simulink model "IEEE_34_node_2020a_scenarios_fold"  (R2020a)
settings: Solver=FixedStepDiscrete  StartTime=0.0  StopTime=0.001  RelTol=1e-3
InitFcn:
  | power_34NodeTestFeeder_init;
  | %=============================
  | Vnom_ph_ph = 24900;
  | Vnom = 24900/sqrt(3);
  | Vnom1_ph_ph = 4160;
  | Vnom1 = 4160/sqrt(3);
  | Degrees_ph_ph_gen1 = 0;
  | Frequency = 60;
  | Apparent_power_gen1 = 2500e3;
  | base_current=1.5e6;
  | SW850_816=1;
  | SW818_820=1;
  | SW832_858=1;
  | SW834_842=1;
  | SW836_862=1;
  | %=============================
  | %824-828===Load1=================
  | V_824_828 = [1.008 1.016 1.012];
  | Pa_824_828 = [1e-6 1e-6 4]*1e3*1;
  | Pp_824_828 = [1e-6 1e-6 2]*1e3*1;
  | Pn_824_828 = [1e-6 1e-6 1e-6]*1;
  | 
  | %820-822===Load2=================
  | V_820_822 = 0.993;
  | Pa_820_822 = 135e3*1;
  | Pp_820_822 = 70e3*1;
  | Pn_820_822 = 1e-6*1;
  | 
  | %858-834===Load3=================
  | V_858_834 = [1.034 1.032 1.034]*sqrt(3);
  | Pa_858_834 = [4 15 13]*1e3*1;
  | Pp_858_834 = [2 8 7]*1e3*1;
  | Pn_858_834 = [1e-6 1e-6 1e-6]*1;
  | 
  | %844 B.V.c===Load4================
  | V_844 = [1.031 1.029 1.031];
  | Pa_844 = [135 135 135]*1e3*1;
  | Pp_844 = [105 105 105]*1e3*1;
  | Pn_844 = [100 100 100]*1e3*1;
  | 
  | %840======Load5=================
  | V_840 = [1.03 1.029 1.031];
  | Pa_840 = [9 9 9]*1e3*1;
  | Pp_840 = [7 7 7]*1e3*1;
  | Pn_840 = [1e-6 1e-6 1e-6]*1;
  | 
  | % For Distributed Loads==================================================
  | %802-806
  | V_802_806 = [1.047 1.048 1.048];
  | Pa_802_806 = [1e-6 30 25]*1e3;
  | Pp_802_806 = [1e-6 15 14]*1e3;
  | Pn_802_806 = [1e-6 1e-6 1e-6];
  | 
  | %808-810
  | V_808_810 = 1.014;
  | Pa_808_810 = 16e3;
  | Pp_808_810 = 8e3;
  | Pn_808_810 = 1e-6;
  | 
  | %816-824
  | V_816_824 = [1.017 1.025 1.02]*sqrt(3);
  | Pa_816_824 = [1e-6 5 1e-6]*1e3;
  | Pp_816_824 = [1e-6 2 1e-6]*1e3;
  | Pn_816_824 = [1e-6 1e-6 1e-6];
  | 
  | %818-820
  | V_818_820 = 1.016;
  | Pa_818_820 = 34e3;
  | Pp_818_820 = 17e3;
  | Pn_818_820 = 1e-6;
  | 
  | %824-826
  | V_824_826 = 1.008;
  | Pa_824_826 = 40e3;
  | Pp_824_826 = 20e3;
  | Pn_824_826 = 1e-6;
  | 
  | %828-830
  | V_828_830 = [1.007 1.015 1.011];
  | Pa_828_830 = [7 1e-6 1e-6]*1e3;
  | Pp_828_830 = [3 1e-6 1e-6]*1e3;
  | Pn_828_830 = [1e-6 1e-6 1e-6];
  | 
  | %832-858
  | V_832_858 = [1.036 1.035 1.036]*sqrt(3);
  | Pa_832_858 = [7 2 6]*1e3;
  | Pp_832_858 = [3 1 3]*1e3;
  | Pn_832_858 = [1e-6 1e-6 1e-6];
  | 
  | %834-860
  | V_834_860 = [1.031 1.029 1.031]*sqrt(3);
  | Pa_834_860 = [16 20 110]*1e3;
  | Pp_834_860 = [8 10 55]*1e3;
  | Pn_834_860 = [1e-6 1e-6 1e-6];
  | 
  | %836-840
  | V_836_840 = [1.03 1.029 1.031]*sqrt(3);
  | Pa_836_840 = [18 22 1e-6]*1e3;
  | Pp_836_840 = [9 11 1e-6]*1e3;
  | Pn_836_840 = [1e-6 1e-6 1e-6];
  | 
  | %842-844
  | V_842_844 = [1.031 1.029 1.031];
  | Pa_842_844 = [9 1e-6 1e-6]*1e3;
  | Pp_842_844 = [5 1e-6 1e-6]*1e3;
  | Pn_842_844 = [1e-6 1e-6 1e-6];
  | 
  | %844-846
  | V_844_846 = [1.031 1.029 1.031];
  | Pa_844_846 = [1e-6 25 20]*1e3;
  | Pp_844_846 = [1e-6 12 11]*1e3;
  | Pn_844_846 = [1e-6 1e-6 1e-6];
  | 
  | %846-848
  | V_846_848 = [1.031 1.029 1.031];
  | Pa_846_848 = [1e-6 23 1e-6]*1e3;
  | Pp_846_848 = [1e-6 11 1e-6]*1e3;
  | Pn_846_848 = [1e-6 1e-6 1e-6];
  | 
  | %854-856
  | V_854_856 = 0.998;
  | Pa_854_856 = 4e3;
  | Pp_854_856 = 2e3;
  | Pn_854_856 = 1e-6;
  | 
  | %858-864
  | V_858_864 = 1.034;
  | Pa_858_864 = 2e3;
  | Pp_858_864 = 1e3;
  | Pn_858_864 = 1e-6;
  | 
  | %860-836
  | V_860_836 = [1.03 1.029 1.031]*sqrt(3);
  | Pa_860_836 = [30 10 42]*1e3;
  | Pp_860_836 = [15 6 22]*1e3;
  | Pn_860_836 = [1e-6 1e-6 1e-6];
  | 
  | %862-838
  | V_862_838 = 1.029;
  | Pa_862_838 = 28e3;
  | Pp_862_838 = 14e3;
  | Pn_862_838 = 1e-6;
  | 
  | % For Spot Loads===========================================================
  | %830
  | V_830 = [0.989 0.998 0.994]*sqrt(3);
  | Pa_830 = [10 10 25]*1e3;
  | Pp_830 = [5 5 10]*1e3;
  | Pn_830 = [1e-6 1e-6 1e-6];
  | 
  | %848 B.V.c
  | V_848 = [1.031 1.029 1.031]*sqrt(3);
  | Pa_848 = [20 20 20]*1e3;
  | Pp_848 = [16 16 16]*1e3;
  | Pn_848 = [150 150 150]*1e3;
  | 
  | %860
  | V_860 = [1.03 1.029 1.031];
  | Pa_860 = [20 20 20]*1e3;
  | Pp_860 = [16 16 16]*1e3;
  | Pn_860 = [1e-6 1e-6 1e-6];
  | 
  | %890
  | V_890 = [0.917 0.924 0.918]*sqrt(3);
  | Pa_890 = [150 150 150]*1e3;
  | Pp_890 = [75 75 75]*1e3;
  | Pn_890 = [1e-6 1e-6 1e-6];
undefined symbols (not defined in the file or in its folder): Angle, C_300, C_301, C_302, C_303, C_304, Degrees_ph, ft2km, L_300, L_301, L_302, L_303, L_304, Magnitude, ph, ph_gen1, R_300, R_301, R_302, R_303, R_304, Vnom_ph
libraries: powerlib x177
(part 1 of 2)
settings Model: Creator=liyifu  LastModifiedBy=l4729
settings DataIOCC: ReturnWorkspaceOutputs=off
settings DebuggingCC: ArithmeticOperatorsInVariantConditions=warning
settings SFSimCC: SimUseLocalCustomCode=off  CustomCodeUndefinedFunction=UseInterfaceOnly
settings RTWCC: RTWUseLocalCustomCode=off

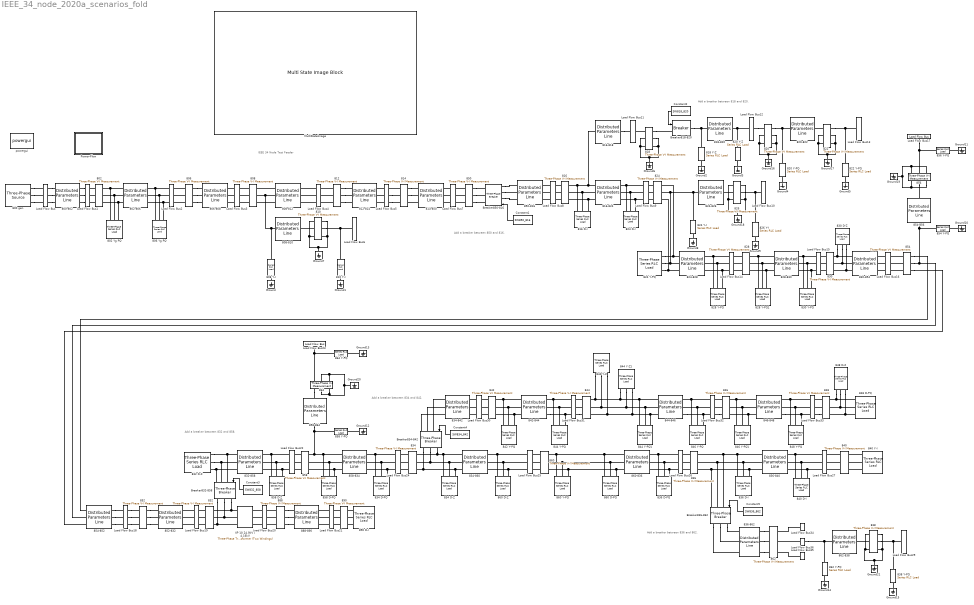
== system IEEE_34_node_2020a_scenarios_fold ==
  note: Add a breaker between 832 and 858.
  note: IEEE 34 Node Test Feeder
  note: Add a breaker between 834 and 842.
  note: Add a breaker between 836 and 862.
  note: Add a breaker between 850 and 816.
  note: Add a breaker between 818 and 820.
  800 gen : powerlib/Electrical Sources/Three-Phase Source  InternalConnection=Yg  VoltagePhases=on  Voltage=Vnom_ph-ph  PhaseAngle=Degrees_ph-ph_gen1  Voltage_phases=[1.05 1.05 1.05]*Vnom  PhaseAngles_phases=[0 -120 +120]  Frequency=Frequency  NonIdealSource=off  SpecifyImpedance=on  Resistance=0.8929  Inductance=16.58e-3  ShortCircuitLevel=Apparent_power_gen1  BaseVoltage=Vnom_ph_ph  XRratio=8  BusType=swing  Pref=10e3  Qref=0  Prefabc=[10e3, 10e3, 10e3]  Qrefabc=[0, 0, 0]  Qmin=-inf  Qmax=inf
  800-802 : powerlib/Elements/Distributed Parameters Line  Phases=3  Frequency=Frequency  Resistance=R_300  Inductance=L_300  Capacitance=C_300  Length=2580*ft2km  x1=[1249.92108084395 26131.4308609001 26009.0181767455;376.991118430775 376.991118430775 376.991118430775;1.94160573810255 0.298080075052811 1.87234868535801]  x2=[1257.86990495326 26107.3117545713 25983.4479681992;376.991118430775 376.991118430775 376.991118430775;1.93807520662352 0.296564075731698 1.87075709202379]  x3=[7.13297479988852 32.3957031974537 23.1415422380633;376.991118430775 376.991118430775 376.991118430775;0.709542259543237 -0.812774214222377 0.255094598667959]  x4=[6.75296406809703 144.806609038061 132.501806105152;376.991118430775 376.991118430775 376.991118430775;-2.86917677084019 0.498468146483693 2.04637828745182]  x5=3.46223763231864e-06  V1=ones(3,3)  V2=ones(3,3)  I1=ones(3,3)  I2=ones(3,3)  nHarmo=1  Measurements=None
  802 : powerlib/Measurements/Three-Phase V-I Measurement  VoltageMeasurement=phase-to-ground  SetLabelV=on  LabelV=Vabc_802  Vpu=on  VpuLL=off  CurrentMeasurement=yes  SetLabelI=on  LabelI=Iabc_802  Ipu=on  Pbase=base_current  Vbase=Vnom_ph_ph  OutputType=Magnitude-Angle  PhasorSimulation=on  PSBequivalent=0
  802 Yg PQ : powerlib/Elements/Three-Phase Series RLC Load  LConnTagsString=A|B|C  Configuration=Y (grounded)  NominalVoltage=[  Vabc=V_802_806*Vnom  Vabcp=[1e3 1e3 1e3]  NominalFrequency=Frequency  UnbalancedPower=on  ActivePower=10e3  InductivePower=100  CapacitivePower=100  Pabc=Pa_802_806/2  QLabc=Pp_802_806/2  QCabc=Pn_802_806  Pabcp=[10e3 9e3 11e3]  QLabcp=[100 90 110]  QCabcp=[100 90 110]  Measurements=None  LoadType=constant PQ
      settings: AttributesFormatString=|
      | P= %<Pabc> W
      | Ql=%<QLabc> var
      | Qc=%<QCabc> var
  802-806 : powerlib/Elements/Distributed Parameters Line  Phases=3  Frequency=Frequency  Resistance=R_300  Inductance=L_300  Capacitance=C_300  Length=1730*ft2km  x1=[1257.86990495326 26107.3117545713 25983.4479681992;376.991118430775 376.991118430775 376.991118430775;1.93850522519394 0.296930576358522 1.87111645643134]  x2=[1263.00777604381 26091.4526622714 25967.1255164436;376.991118430775 376.991118430775 376.991118430775;1.93674169452962 0.295921998479355 1.87004589016608]  x3=[6.73268295673131 32.7537595825314 24.3418370556638;376.991118430775 376.991118430775 376.991118430775;0.817345362469665 -0.791135380998958 0.306817144760857]  x4=[6.06072552939003 143.954163081489 131.457799242515;376.991118430775 376.991118430775 376.991118430775;-2.79432744429802 0.498877931254703 2.05645367118062]  x5=2.32157794725242e-06  V1=ones(3,3)  V2=ones(3,3)  I1=ones(3,3)  I2=ones(3,3)  nHarmo=1  Measurements=None
  806 : powerlib/Measurements/Three-Phase V-I Measurement  VoltageMeasurement=phase-to-ground  SetLabelV=on  LabelV=Vabc_806  Vpu=on  VpuLL=off  CurrentMeasurement=yes  SetLabelI=on  LabelI=Iabc_806  Ipu=on  Pbase=base_current  Vbase=Vnom_ph_ph  OutputType=Magnitude-Angle  PhasorSimulation=on  PSBequivalent=0
  806 Yg PQ : powerlib/Elements/Three-Phase Series RLC Load  LConnTagsString=A|B|C  Configuration=Y (grounded)  NominalVoltage=[  Vabc=V_802_806*Vnom  Vabcp=[1e3 1e3 1e3]  NominalFrequency=Frequency  UnbalancedPower=on  ActivePower=10e3  InductivePower=100  CapacitivePower=100  Pabc=Pa_802_806/2  QLabc=Pp_802_806/2  QCabc=Pn_802_806  Pabcp=[10e3 9e3 11e3]  QLabcp=[100 90 110]  QCabcp=[100 90 110]  Measurements=None  LoadType=constant PQ
      settings: AttributesFormatString=|
      | P= %<Pabc> W
      | Ql=%<QLabc> var
      | Qc=%<QCabc> var
  806-808 : powerlib/Elements/Distributed Parameters Line  Phases=3  Frequency=Frequency  Resistance=R_300  Inductance=L_300  Capacitance=C_300  Length=32230*ft2km  x1=[1263.00777604381 26091.4526622714 25967.1255164436;376.991118430775 376.991118430775 376.991118430775;1.92131161641447 0.282771093634514 1.85715104965965]  x2=[1355.16892465068 25803.6960566382 25680.9632225794;376.991118430775 376.991118430775 376.991118430775;1.90095381776325 0.264070563711962 1.8370468229557]  x3=[6.3768548007228 32.6175711680747 25.3697798294854;376.991118430775 376.991118430775 376.991118430775;0.920439308030638 -0.792962958654931 0.330886039817891]  x4=[5.31865755565328 140.041353428377 128.050295750342;376.991118430775 376.991118430775 376.991118430775;-2.73456087382505 0.471033237587638 2.03937541131982]  x5=4.32511313525697e-05  V1=ones(3,3)  V2=ones(3,3)  I1=ones(3,3)  I2=ones(3,3)  nHarmo=1  Measurements=None
  808 : powerlib/Measurements/Three-Phase V-I Measurement  VoltageMeasurement=phase-to-ground  SetLabelV=on  LabelV=Vabc_808  Vpu=on  VpuLL=off  CurrentMeasurement=yes  SetLabelI=on  LabelI=Iabc_808  Ipu=on  Pbase=base_current  Vbase=Vnom_ph_ph  OutputType=Magnitude-Angle  PhasorSimulation=on  PSBequivalent=0
  808 Y-I : powerlib/Elements/Series RLC Load  LConnTagsString=a  RConnTagsString=__new0  NominalVoltage=V_808_810*Vnom  NominalFrequency=Frequency  ActivePower=Pa_808_810/2  InductivePower=Pp_808_810/2  CapacitivePower=Pn_808_810  Setx0=off  InitialVoltage=0  SetiL0=off  InitialCurrent=0  Measurements=None  LoadType=constant I
      settings: AttributesFormatString=|
      | P=%<ActivePower> W
      | Ql=%<InductivePower> var
      | Qc=%<CapacitivePower> var
  808-810 : powerlib/Elements/Distributed Parameters Line  Phases=1  Frequency=Frequency  Resistance=R_303(2,2)  Inductance=L_303(2,2)  Capacitance=C_303(2,2)  Length=5804*ft2km  x1=[21047.5384749886;376.991118430775;-2.12176362657333]  x2=[21044.5333181041;376.991118430775;-2.12177432032583]  x3=[34.5695272211914;376.991118430775;-2.11315403228961]  x4=[36.1457970114117;376.991118430775;-2.13270557006442]  x5=7.30496713110932e-06  V1=ones(3,3)  V2=ones(3,3)  I1=ones(3,3)  I2=ones(3,3)  nHarmo=1  Measurements=None
  808-812 : powerlib/Elements/Distributed Parameters Line  Phases=3  Frequency=Frequency  Resistance=R_300  Inductance=L_300  Capacitance=C_300  Length=37500*ft2km  x1=[1355.16892465068 25803.6960566382 25680.9632225794;376.991118430775 376.991118430775 376.991118430775;1.89828770262664 0.261798259825657 1.83481876362885]  x2=[1443.44628212571 25479.8515014695 25364.0620665995;376.991118430775 376.991118430775 376.991118430775;1.88295137638678 0.240192551529379 1.81094740401628]  x3=[5.46905993850028 32.6245925749511 26.6761925732301;376.991118430775 376.991118430775 376.991118430775;0.995018334108287 -0.794161100185234 0.309761347978168]  x4=[4.23685935060835 137.208461244538 126.419269863165;376.991118430775 376.991118430775 376.991118430775;-2.8061655132456 0.449094607298641 2.02713913226157]  x5=5.03232213999802e-05  V1=ones(3,3)  V2=ones(3,3)  I1=ones(3,3)  I2=ones(3,3)  nHarmo=1  Measurements=None
  810 : powerlib/Measurements/Three-Phase V-I Measurement  VoltageMeasurement=phase-to-ground  SetLabelV=on  LabelV=Vabc_810  Vpu=on  VpuLL=off  CurrentMeasurement=yes  SetLabelI=on  LabelI=Iabc_810  Ipu=on  Pbase=base_current  Vbase=Vnom_ph_ph  OutputType=Magnitude-Angle  PhasorSimulation=on  PSBequivalent=0
  810 Y-I : powerlib/Elements/Series RLC Load  LConnTagsString=a  RConnTagsString=__new0  NominalVoltage=V_808_810*Vnom  NominalFrequency=Frequency  ActivePower=Pa_808_810/2  InductivePower=Pp_808_810/2  CapacitivePower=Pn_808_810  Setx0=off  InitialVoltage=0  SetiL0=off  InitialCurrent=0  Measurements=None  LoadType=constant I
      settings: AttributesFormatString=|
      | P=%<ActivePower> W
      | Ql=%<InductivePower> var
      | Qc=%<CapacitivePower> var
  812 : powerlib/Measurements/Three-Phase V-I Measurement  VoltageMeasurement=phase-to-ground  SetLabelV=on  LabelV=Vabc_812  Vpu=on  VpuLL=off  CurrentMeasurement=yes  SetLabelI=on  LabelI=Iabc_812  Ipu=on  Pbase=base_current  Vbase=Vnom_ph_ph  OutputType=Magnitude-Angle  PhasorSimulation=on  PSBequivalent=0
  812-814 : powerlib/Elements/Distributed Parameters Line  Phases=3  Frequency=Frequency  Resistance=R_300  Inductance=L_300  Capacitance=C_300  Length=29730*ft2km  x1=[1443.44628212571 25479.8515014695 25364.0620665995;376.991118430775 376.991118430775 376.991118430775;1.88688225202464 0.243542798435754 1.814232417483]  x2=[1513.27779103294 25226.8818502461 25118.6711360678;376.991118430775 376.991118430775 376.991118430775;1.87617344887056 0.226298980649994 1.79510755585285]  x3=[5.53984525286875 32.6362598627681 27.1978990110373;376.991118430775 376.991118430775 376.991118430775;1.01474929706559 -0.819913423956052 0.285686013441521]  x4=[4.19567507962093 136.436942339818 125.720705102048;376.991118430775 376.991118430775 376.991118430775;-2.82219411836218 0.437343389389646 2.01609371330485]  x5=3.98962499259043e-05  V1=ones(3,3)  V2=ones(3,3)  I1=ones(3,3)  I2=ones(3,3)  nHarmo=1  Measurements=None
  814 : powerlib/Measurements/Three-Phase V-I Measurement  VoltageMeasurement=phase-to-ground  SetLabelV=on  LabelV=Vabc_814  Vpu=on  VpuLL=off  CurrentMeasurement=yes  SetLabelI=on  LabelI=Iabc_814  Ipu=on  Pbase=base_current  Vbase=Vnom_ph_ph  OutputType=Magnitude-Angle  PhasorSimulation=on  PSBequivalent=0
  814-850 : powerlib/Elements/Distributed Parameters Line  Phases=3  Frequency=Frequency  Resistance=R_301  Inductance=L_301  Capacitance=C_301  Length=10*ft2km  x1=[749.994335266099 25229.1164810927 25142.5492609672;376.991118430775 376.991118430775 376.991118430775;-0.624184699531901 0.237600670627926 1.80412447902211]  x2=[749.971210173394 25228.9677045473 25142.4037426608;376.991118430775 376.991118430775 376.991118430775;-0.624161374265916 0.237593581391487 1.80411674762356]  x3=[4.46442861433734 31.9624950383377 28.1850985340397;376.991118430775 376.991118430775 376.991118430775;0.862042492492586 -0.884382499448575 0.236346932718508]  x4=[4.62367269240938 136.132716168199 125.203043967645;376.991118430775 376.991118430775 376.991118430775;-1.91880432400362 0.45074101824152 2.03117866069587]  x5=1.37899021776565e-08  V1=ones(3,3)  V2=ones(3,3)  I1=ones(3,3)  I2=ones(3,3)  nHarmo=1  Measurements=None
  816 : powerlib/Measurements/Three-Phase V-I Measurement  VoltageMeasurement=phase-to-ground  SetLabelV=on  LabelV=Vabc_816  Vpu=on  VpuLL=off  CurrentMeasurement=yes  SetLabelI=on  LabelI=Iabc_816  Ipu=on  Pbase=base_current  Vbase=Vnom_ph_ph  OutputType=Magnitude-Angle  PhasorSimulation=on  PSBequivalent=0
  816 D-I : powerlib/Elements/Three-Phase Series RLC Load  LConnTagsString=A|B|C  Configuration=Delta  NominalVoltage=[  Vabc=[1.017 1.025 1.02]*sqrt(3)*Vnom  Vabcp=V_816_824*Vnom  NominalFrequency=Frequency  UnbalancedPower=on  ActivePower=10e3  InductivePower=100  CapacitivePower=100  Pabc=[0 30 25]*1e3/2  QLabc=[0 15 14]*1e3/2  QCabc=[0 0 0]  Pabcp=Pa_816_824/2  QLabcp=Pp_816_824/2  QCabcp=Pn_816_824  Measurements=None  LoadType=constant I
      settings: AttributesFormatString=|
      | P= %<Pabc> W
      | Ql=%<QLabc> var
      | Qc=%<QCabc> var
  816-818 : powerlib/Elements/Distributed Parameters Line  Phases=1  Frequency=Frequency  Resistance=R_302(1,1)  Inductance=L_302(1,1)  Capacitance=C_302(1,1)  Length=1710*ft2km  x1=[20492.3335751348;376.991118430775;-0.0532831391288457]  x2=[20492.3403203766;376.991118430775;-0.05328375944644]  x3=[34.5203913919803;376.991118430775;-0.0540948176909164]  x4=[34.5203913965351;376.991118430775;-0.053283759447173]  x5=2.15222153587128e-06  V1=ones(3,3)  V2=ones(3,3)  I1=ones(3,3)  I2=ones(3,3)  nHarmo=1  Measurements=None
  816-824 : powerlib/Elements/Distributed Parameters Line  Phases=3  Frequency=Frequency  Resistance=R_301  Inductance=L_301  Capacitance=C_301  Length=10210*ft2km  x1=[749.254552412163 25224.3500731886 25137.8871613909;376.991118430775 376.991118430775 376.991118430775;-0.62873965530836 0.233052102249028 1.79962312608389]  x2=[725.798891896366 25072.9462538103 24990.6123339841;376.991118430775 376.991118430775 376.991118430775;-0.604102731040263 0.225801070087458 1.79169218001229]  x3=[4.45992554408711 31.6940310924998 28.2049487981477;376.991118430775 376.991118430775 376.991118430775;0.859034713727634 -0.891901311045086 0.232740974635364]  x4=[4.59825263303408 134.634587751809 123.946758724965;376.991118430775 376.991118430775 376.991118430775;-1.92767802301581 0.440691491205759 2.02309252339209]  x5=1.40794901233873e-05  V1=ones(3,3)  V2=ones(3,3)  I1=ones(3,3)  I2=ones(3,3)  nHarmo=1  Measurements=None
  818 : powerlib/Measurements/Three-Phase V-I Measurement  VoltageMeasurement=phase-to-ground  SetLabelV=on  LabelV=Vabc_818  Vpu=on  VpuLL=off  CurrentMeasurement=yes  SetLabelI=on  LabelI=Iabc_818  Ipu=on  Pbase=base_current  Vbase=Vnom_ph_ph  OutputType=Magnitude-Angle  PhasorSimulation=on  PSBequivalent=0
  818 Y-Z : powerlib/Elements/Series RLC Load  LConnTagsString=a  RConnTagsString=__new0  NominalVoltage=V_818_820*Vnom  NominalFrequency=Frequency  ActivePower=Pa_818_820/2  InductivePower=Pp_818_820/2  CapacitivePower=Pn_818_820  Setx0=off  InitialVoltage=0  SetiL0=off  InitialCurrent=0  Measurements=None  LoadType=constant Z
      settings: AttributesFormatString=|
      | P=%<ActivePower> W
      | Ql=%<InductivePower> var
      | Qc=%<CapacitivePower> var
  818-820 : powerlib/Elements/Distributed Parameters Line  Phases=1  Frequency=Frequency  Resistance=R_302(1,1)  Inductance=L_302(1,1)  Capacitance=C_302(1,1)  Length=48150*ft2km  x1=[3.14486863470603e-11;376.991118430775;-0.211800871501961]  x2=[2.45219954924631e-11;376.991118430775;-0.489738438513156]  x3=[3.00836533610094e-13;376.991118430775;-3.09485858385258]  x4=[3.86066249532496e-13;376.991118430775;-0.0429229789502031]  x5=6.06020274574283e-05  V1=ones(3,3)  V2=ones(3,3)  I1=ones(3,3)  I2=ones(3,3)  nHarmo=1  Measurements=None
  820 : powerlib/Measurements/Three-Phase V-I Measurement  VoltageMeasurement=phase-to-ground  SetLabelV=on  LabelV=Vabc_820  Vpu=on  VpuLL=off  CurrentMeasurement=yes  SetLabelI=on  LabelI=Iabc_820  Ipu=on  Pbase=base_current  Vbase=Vnom_ph_ph  OutputType=Magnitude-Angle  PhasorSimulation=on  PSBequivalent=0
  820 Y-PQ : powerlib/Elements/Series RLC Load  LConnTagsString=a  RConnTagsString=__new0  NominalVoltage=V_820_822*Vnom  NominalFrequency=Frequency  ActivePower=Pa_820_822/2  InductivePower=Pp_820_822/2  CapacitivePower=Pn_820_822  Setx0=off  InitialVoltage=0  SetiL0=off  InitialCurrent=0  Measurements=None  LoadType=constant PQ
      settings: AttributesFormatString=|
      | P=%<ActivePower> W
      | Ql=%<InductivePower> var
      | Qc=%<CapacitivePower> var
  820 Y-Z : powerlib/Elements/Series RLC Load  LConnTagsString=a  RConnTagsString=__new0  NominalVoltage=V_818_820*Vnom  NominalFrequency=Frequency  ActivePower=Pa_818_820/2  InductivePower=Pp_818_820/2  CapacitivePower=Pn_818_820  Setx0=off  InitialVoltage=0  SetiL0=off  InitialCurrent=0  Measurements=None  LoadType=constant Z
      settings: AttributesFormatString=|
      | P=%<ActivePower> W
      | Ql=%<InductivePower> var
      | Qc=%<CapacitivePower> var
  820-822 : powerlib/Elements/Distributed Parameters Line  Phases=1  Frequency=Frequency  Resistance=R_302(1,1)  Inductance=L_302(1,1)  Capacitance=C_302(1,1)  Length=13740*ft2km  x1=[2.45219954924631e-11;376.991118430775;-0.473411428700963]  x2=[2.44472924380302e-11;376.991118430775;-0.47348054014256]  x3=[3.31598968730564e-14;376.991118430775;-0.355342569806625]  x4=[4.90777691211079e-14;376.991118430775;-0.558612938007749]  x5=1.72932888320886e-05  V1=ones(3,3)  V2=ones(3,3)  I1=ones(3,3)  I2=ones(3,3)  nHarmo=1  Measurements=None
  822 : powerlib/Measurements/Three-Phase V-I Measurement  VoltageMeasurement=phase-to-ground  SetLabelV=on  LabelV=Vabc_822  Vpu=on  VpuLL=off  CurrentMeasurement=yes  SetLabelI=on  LabelI=Iabc_822  Ipu=on  Pbase=base_current  Vbase=Vnom_ph_ph  OutputType=Magnitude-Angle  PhasorSimulation=on  PSBequivalent=0
  822 Y-PQ : powerlib/Elements/Series RLC Load  LConnTagsString=a  RConnTagsString=__new0  NominalVoltage=V_820_822*Vnom  NominalFrequency=Frequency  ActivePower=Pa_820_822/2  InductivePower=Pp_820_822/2  CapacitivePower=Pn_820_822  Setx0=off  InitialVoltage=0  SetiL0=off  InitialCurrent=0  Measurements=None  LoadType=constant PQ
      settings: AttributesFormatString=|
      | P=%<ActivePower> W
      | Ql=%<InductivePower> var
      | Qc=%<CapacitivePower> var
  824 : powerlib/Measurements/Three-Phase V-I Measurement  VoltageMeasurement=phase-to-ground  SetLabelV=on  LabelV=Vabc_824  Vpu=on  VpuLL=off  CurrentMeasurement=yes  SetLabelI=on  LabelI=Iabc_824  Ipu=on  Pbase=base_current  Vbase=Vnom_ph_ph  OutputType=Magnitude-Angle  PhasorSimulation=on  PSBequivalent=0
  824 D-I : powerlib/Elements/Three-Phase Series RLC Load  LConnTagsString=A|B|C  Configuration=Delta  NominalVoltage=[  Vabc=[1.017 1.025 1.02]*sqrt(3)*Vnom  Vabcp=V_816_824*Vnom  NominalFrequency=Frequency  UnbalancedPower=on  ActivePower=10e3  InductivePower=100  CapacitivePower=100  Pabc=[0 30 25]*1e3/2  QLabc=[0 15 14]*1e3/2  QCabc=[0 0 0]  Pabcp=Pa_816_824/2  QLabcp=Pp_816_824/2  QCabcp=Pn_816_824  Measurements=None  LoadType=constant I
      settings: AttributesFormatString=|
      | P= %<Pabc> W
      | Ql=%<QLabc> var
      | Qc=%<QCabc> var
  824 Y-I : powerlib/Elements/Series RLC Load  LConnTagsString=a  RConnTagsString=__new0  NominalVoltage=V_824_826*Vnom  NominalFrequency=Frequency  ActivePower=Pa_824_826/2  InductivePower=Pp_824_826/2  CapacitivePower=Pn_824_826  Setx0=off  InitialVoltage=0  SetiL0=off  InitialCurrent=0  Measurements=None  LoadType=constant I
      settings: AttributesFormatString=|
      | P=%<ActivePower> W
      | Ql=%<InductivePower> var
      | Qc=%<CapacitivePower> var
  824 Y-PQ : powerlib/Elements/Three-Phase Series RLC Load  LConnTagsString=A|B|C  Configuration=Y (grounded)  NominalVoltage=[  Vabc=V_824_828*Vnom  Vabcp=[1.008 1.016 1.012]*Vnom  NominalFrequency=Frequency  UnbalancedPower=on  ActivePower=10e3  InductivePower=100  CapacitivePower=100  Pabc=Pa_824_828/2  QLabc=Pp_824_828/2  QCabc=Pn_824_828  Pabcp=[0 0 4]*1e3/2  QLabcp=[0 0 2]*1e3/2  QCabcp=[0 0 0]  Measurements=None  LoadType=constant PQ
      settings: AttributesFormatString=|
      | P= %<Pabc> W
      | Ql=%<QLabc> var
      | Qc=%<QCabc> var
  824-826 : powerlib/Elements/Distributed Parameters Line  Phases=1  Frequency=Frequency  Resistance=R_303(2,2)  Inductance=L_303(2,2)  Capacitance=C_303(2,2)  Length=3030*ft2km  x1=[20431.4343856754;376.991118430775;-2.17401677873248]  x2=[20427.5005961486;376.991118430775;-2.17402341201917]  x3=[32.4575119217889;376.991118430775;-2.14560616936423]  x4=[36.3366460329366;376.991118430775;-2.20076180502658]  x5=3.81358552847368e-06  V1=ones(3,3)  V2=ones(3,3)  I1=ones(3,3)  I2=ones(3,3)  nHarmo=1  Measurements=None
  824-828 : powerlib/Elements/Distributed Parameters Line  Phases=3  Frequency=Frequency  Resistance=R_301  Inductance=L_301  Capacitance=C_301  Length=840*ft2km  x1=[725.798891896366 25072.9462538104 24990.6123339841;376.991118430775 376.991118430775 376.991118430775;-0.599231576645892 0.229770989630034 1.79559984451946]  x2=[724.333204252172 25061.125944867 24979.1581902396;376.991118430775 376.991118430775 376.991118430775;-0.598937094945461 0.229192975042994 1.79492479353475]  x3=[2.36107488025287 32.4318859411575 30.9455826644874;376.991118430775 376.991118430775 376.991118430775;1.29350978989862 -0.817216623978334 0.25983718422928]  x4=[3.23206893655298 132.662549876552 124.067629122138;376.991118430775 376.991118430775 376.991118430775;-1.36489767846073 0.442550200247547 2.04701107148014]  x5=1.15835178292315e-06  V1=ones(3,3)  V2=ones(3,3)  I1=ones(3,3)  I2=ones(3,3)  nHarmo=1  Measurements=None
  826 : powerlib/Measurements/Three-Phase V-I Measurement  VoltageMeasurement=phase-to-ground  SetLabelV=on  LabelV=Vabc_826  Vpu=on  VpuLL=off  CurrentMeasurement=yes  SetLabelI=on  LabelI=Iabc_826  Ipu=on  Pbase=base_current  Vbase=Vnom_ph_ph  OutputType=Magnitude-Angle  PhasorSimulation=on  PSBequivalent=0
  826 Y-I : powerlib/Elements/Series RLC Load  LConnTagsString=a  RConnTagsString=__new0  NominalVoltage=V_824_826*Vnom  NominalFrequency=Frequency  ActivePower=Pa_824_826/2  InductivePower=Pp_824_826/2  CapacitivePower=Pn_824_826  Setx0=off  InitialVoltage=0  SetiL0=off  InitialCurrent=0  Measurements=None  LoadType=constant I
      settings: AttributesFormatString=|
      | P=%<ActivePower> W
      | Ql=%<InductivePower> var
      | Qc=%<CapacitivePower> var
  828 : powerlib/Measurements/Three-Phase V-I Measurement  VoltageMeasurement=phase-to-ground  SetLabelV=on  LabelV=Vabc_828  Vpu=on  VpuLL=off  CurrentMeasurement=yes  SetLabelI=on  LabelI=Iabc_828  Ipu=on  Pbase=base_current  Vbase=Vnom_ph_ph  OutputType=Magnitude-Angle  PhasorSimulation=on  PSBequivalent=0
  828 Y-PQ : powerlib/Elements/Three-Phase Series RLC Load  LConnTagsString=A|B|C  Configuration=Y (grounded)  NominalVoltage=[  Vabc=V_824_828*Vnom  Vabcp=[1.008 1.016 1.012]*Vnom  NominalFrequency=Frequency  UnbalancedPower=on  ActivePower=10e3  InductivePower=100  CapacitivePower=100  Pabc=Pa_824_828/2  QLabc=Pp_824_828/2  QCabc=Pn_824_828  Pabcp=[0 0 4]*1e3/2  QLabcp=[0 0 2]*1e3/2  QCabcp=[0 0 0]  Measurements=None  LoadType=constant PQ
      settings: AttributesFormatString=|
      | P= %<Pabc> W
      | Ql=%<QLabc> var
      | Qc=%<QCabc> var
  828 Y-PQ1 : powerlib/Elements/Three-Phase Series RLC Load  LConnTagsString=A|B|C  Configuration=Y (grounded)  NominalVoltage=[  Vabc=V_828_830*Vnom  Vabcp=[1.008 1.016 1.012]*Vnom  NominalFrequency=Frequency  UnbalancedPower=on  ActivePower=10e3  InductivePower=100  CapacitivePower=100  Pabc=Pa_828_830/2  QLabc=Pp_828_830/2  QCabc=Pn_828_830  Pabcp=[0 0 4]*1e3/2  QLabcp=[0 0 2]*1e3/2  QCabcp=[0 0 0]  Measurements=None  LoadType=constant PQ
      settings: AttributesFormatString=|
      | P= %<Pabc> W
      | Ql=%<QLabc> var
      | Qc=%<QCabc> var
  828-830 : powerlib/Elements/Distributed Parameters Line  Phases=3  Frequency=Frequency  Resistance=R_301  Inductance=L_301  Capacitance=C_301  Length=20440*ft2km  x1=[724.333204252172 25061.125944867 24979.1581902396;376.991118430775 376.991118430775 376.991118430775;-0.609126489409672 0.220888767675387 1.78675081014729]  x2=[688.850996548628 24777.1500845193 24704.4070912414;376.991118430775 376.991118430775 376.991118430775;-0.597582089374653 0.206708269291752 1.77024155283466]  x3=[2.43064340571967 32.2644476147078 30.7106760769254;376.991118430775 376.991118430775 376.991118430775;1.20592518919778 -0.833386025515453 0.250647142449248]  x4=[3.17065339409325 129.832477428634 121.675601572527;376.991118430775 376.991118430775 376.991118430775;-1.44772404503621 0.42584762229397 2.02913027749089]  x5=2.81865600511299e-05  V1=ones(3,3)  V2=ones(3,3)  I1=ones(3,3)  I2=ones(3,3)  nHarmo=1  Measurements=None
  830 : powerlib/Measurements/Three-Phase V-I Measurement  VoltageMeasurement=phase-to-ground  SetLabelV=on  LabelV=Vabc_830  Vpu=on  VpuLL=off  CurrentMeasurement=yes  SetLabelI=on  LabelI=Iabc_830  Ipu=on  Pbase=base_current  Vbase=Vnom_ph_ph  OutputType=Magnitude-Angle  PhasorSimulation=on  PSBequivalent=0
  830 D-Z : powerlib/Elements/Three-Phase Series RLC Load  LConnTagsString=A|B|C  Configuration=Delta  NominalVoltage=[  Vabc=[1.017 1.025 1.02]*sqrt(3)*Vnom  Vabcp=V_830*Vnom  NominalFrequency=Frequency  UnbalancedPower=on  ActivePower=10e3  InductivePower=100  CapacitivePower=100  Pabc=[0 30 25]*1e3/2  QLabc=[0 15 14]*1e3/2  QCabc=[0 0 0]  Pabcp=Pa_830  QLabcp=Pp_830  QCabcp=Pn_830  Measurements=None  LoadType=constant Z
      settings: AttributesFormatString=|
      | P= %<Pabc> W
      | Ql=%<QLabc> var
      | Qc=%<QCabc> var
  830 Y-PQ : powerlib/Elements/Three-Phase Series RLC Load  LConnTagsString=A|B|C  Configuration=Y (grounded)  NominalVoltage=[  Vabc=V_828_830*Vnom  Vabcp=[1.008 1.016 1.012]*Vnom  NominalFrequency=Frequency  UnbalancedPower=on  ActivePower=10e3  InductivePower=100  CapacitivePower=100  Pabc=Pa_828_830/2  QLabc=Pp_828_830/2  QCabc=Pn_828_830  Pabcp=[0 0 4]*1e3/2  QLabcp=[0 0 2]*1e3/2  QCabcp=[0 0 0]  Measurements=None  LoadType=constant PQ
      settings: AttributesFormatString=|
      | P= %<Pabc> W
      | Ql=%<QLabc> var
      | Qc=%<QCabc> var
  830-854 : powerlib/Elements/Distributed Parameters Line  Phases=3  Frequency=Frequency  Resistance=R_301  Inductance=L_301  Capacitance=C_301  Length=520*ft2km  x1=[688.850996548628 24777.1500845193 24704.4070912414;376.991118430775 376.991118430775 376.991118430775;-0.587226337449802 0.215148055555157 1.77854898901212]  x2=[688.035917811594 24770.3844862052 24697.8456577878;376.991118430775 376.991118430775 376.991118430775;-0.586812515383665 0.21478012546936 1.77813256606496]  x3=[2.36219795478491 34.9317374837201 31.7157275561844;376.991118430775 376.991118430775 376.991118430775;1.09793938051101 -0.821340557343332 0.310858993675246]  x4=[2.94101523771982 129.944451583915 120.813336931978;376.991118430775 376.991118430775 376.991118430775;-1.51104201945579 0.448280427637253 2.04241017587688]  x5=7.17074913238139e-07  V1=ones(3,3)  V2=ones(3,3)  I1=ones(3,3)  I2=ones(3,3)  nHarmo=1  Measurements=None
  832 : powerlib/Measurements/Three-Phase V-I Measurement  VoltageMeasurement=phase-to-ground  SetLabelV=on  LabelV=Vabc_832  Vpu=on  VpuLL=off  CurrentMeasurement=yes  SetLabelI=on  LabelI=Iabc_832  Ipu=on  Pbase=base_current  Vbase=Vnom_ph_ph  OutputType=Magnitude-Angle  PhasorSimulation=on  PSBequivalent=0
  832 D-Z : powerlib/Elements/Three-Phase Series RLC Load  LConnTagsString=A|B|C  Configuration=Delta  NominalVoltage=[  Vabc=[1.017 1.025 1.02]*sqrt(3)*Vnom  Vabcp=V_832_858*Vnom  NominalFrequency=Frequency  UnbalancedPower=on  ActivePower=10e3  InductivePower=100  CapacitivePower=100  Pabc=[0 30 25]*1e3/2  QLabc=[0 15 14]*1e3/2  QCabc=[0 0 0]  Pabcp=Pa_832_858/2  QLabcp=Pp_832_858/2  QCabcp=Pn_832_858  Measurements=None  LoadType=constant Z
      settings: AttributesFormatString=|
      | P= %<Pabc> W
      | Ql=%<QLabc> var
      | Qc=%<QCabc> var
  832-858 : powerlib/Elements/Distributed Parameters Line  Phases=3  Frequency=Frequency  Resistance=R_301  Inductance=L_301  Capacitance=C_301  Length=4900*ft2km  x1=[636.228363410345 24296.443859695 24244.1315726922;376.991118430775 376.991118430775 376.991118430775;-0.560461161079687 0.186755978164699 1.74647760957454]  x2=[632.750499487762 24270.3723308237 24221.7201740198;376.991118430775 376.991118430775 376.991118430775;-0.556682388337997 0.183129201053796 1.74244364860058]  x3=[1.40533220299071 53.6723513113573 47.5031962264219;376.991118430775 376.991118430775 376.991118430775;0.645235196803292 -0.659736273662097 0.641414583104401]  x4=[1.58048483682928 112.631735845984 104.813461005557;376.991118430775 376.991118430775 376.991118430775;-1.53963483994723 0.547888374514142 2.15967981395581]  x5=6.7570520670517e-06  V1=ones(3,3)  V2=ones(3,3)  I1=ones(3,3)  I2=ones(3,3)  nHarmo=1  Measurements=None
  834 : powerlib/Measurements/Three-Phase V-I Measurement  VoltageMeasurement=phase-to-ground  SetLabelV=on  LabelV=Vabc_834  Vpu=on  VpuLL=off  CurrentMeasurement=yes  SetLabelI=on  LabelI=Iabc_834  Ipu=on  Pbase=base_current  Vbase=Vnom_ph_ph  OutputType=Magnitude-Angle  PhasorSimulation=on  PSBequivalent=0
  834 D-PQ : powerlib/Elements/Three-Phase Series RLC Load  LConnTagsString=A|B|C  Configuration=Delta  NominalVoltage=[  Vabc=[1.017 1.025 1.02]*sqrt(3)*Vnom  Vabcp=V_858_834*Vnom  NominalFrequency=Frequency  UnbalancedPower=on  ActivePower=10e3  InductivePower=100  CapacitivePower=100  Pabc=[0 30 25]*1e3/2  QLabc=[0 15 14]*1e3/2  QCabc=[0 0 0]  Pabcp=Pa_858_834/2  QLabcp=Pp_858_834/2  QCabcp=Pn_858_834  Measurements=None  LoadType=constant PQ
      settings: AttributesFormatString=|
      | P= %<Pabc> W
      | Ql=%<QLabc> var
      | Qc=%<QCabc> var
  834 D-Z : powerlib/Elements/Three-Phase Series RLC Load  LConnTagsString=A|B|C  Configuration=Delta  NominalVoltage=[  Vabc=[1.017 1.025 1.02]*sqrt(3)*Vnom  Vabcp=V_834_860*Vnom  NominalFrequency=Frequency  UnbalancedPower=on  ActivePower=10e3  InductivePower=100  CapacitivePower=100  Pabc=[0 30 25]*1e3/2  QLabc=[0 15 14]*1e3/2  QCabc=[0 0 0]  Pabcp=Pa_834_860/2  QLabcp=Pp_834_860/2  QCabcp=Pn_834_860  Measurements=None  LoadType=constant Z
      settings: AttributesFormatString=|
      | P= %<Pabc> W
      | Ql=%<QLabc> var
      | Qc=%<QCabc> var
  834-842 : powerlib/Elements/Distributed Parameters Line  Phases=3  Frequency=Frequency  Resistance=R_301  Inductance=L_301  Capacitance=C_301  Length=280*ft2km  x1=[629.097809541798 24241.627177362 24197.7554674512;376.991118430775 376.991118430775 376.991118430775;-0.549199058758925 0.180761387933223 1.73958434740176]  x2=[629.171950440656 24241.8892384644 24198.3112498873;376.991118430775 376.991118430775 376.991118430775;-0.549397546599232 0.180537220425316 1.73936515346356]  x3=[0.893695246196905 71.7728433905162 62.1894919194319;376.991118430775 376.991118430775 376.991118430775;-1.58010765146336 -0.616677578114269 0.839897927734232]  x4=[1.19309533637291 104.487858505106 92.6235053568442;376.991118430775 376.991118430775 376.991118430775;0.148318450138134 0.694336216295322 2.29300369240257]  x5=3.86117260974383e-07  V1=ones(3,3)  V2=ones(3,3)  I1=ones(3,3)  I2=ones(3,3)  nHarmo=1  Measurements=None
  834-860 : powerlib/Elements/Distributed Parameters Line  Phases=3  Frequency=Frequency  Resistance=R_301  Inductance=L_301  Capacitance=C_301  Length=2020*ft2km  x1=[629.097777973359 24241.6292315875 24197.757448572;376.991118430775 376.991118430775 376.991118430775;-0.550103539411176 0.180024389295677 1.73885889792105]  x2=[627.6711248122 24232.0625215145 24188.4434896558;376.991118430775 376.991118430775 376.991118430775;-0.546824540148702 0.180084266752046 1.73884465023947]  x3=[2.16560598280331 59.5396049892757 47.5719546908952;376.991118430775 376.991118430775 376.991118430775;0.48900550141419 0.304642524618513 1.85714215242525]  x4=[1.88505506572763 82.205536839596 70.3173661655052;376.991118430775 376.991118430775 376.991118430775;-1.9753561544694 0.0891921722452065 1.65822061298159]  x5=2.78556023988662e-06  V1=ones(3,3)  V2=ones(3,3)  I1=ones(3,3)  I2=ones(3,3)  nHarmo=1  Measurements=None
  836 : powerlib/Measurements/Three-Phase V-I Measurement  VoltageMeasurement=phase-to-ground  SetLabelV=on  LabelV=Vabc_836  Vpu=on  VpuLL=off  CurrentMeasurement=yes  SetLabelI=on  LabelI=Iabc_836  Ipu=on  Pbase=base_current  Vbase=Vnom_ph_ph  OutputType=Magnitude-Angle  PhasorSimulation=on  PSBequivalent=0
  836 D-I : powerlib/Elements/Three-Phase Series RLC Load  LConnTagsString=A|B|C  Configuration=Delta  NominalVoltage=[  Vabc=[1.017 1.025 1.02]*sqrt(3)*Vnom  Vabcp=V_836_840*Vnom  NominalFrequency=Frequency  UnbalancedPower=on  ActivePower=10e3  InductivePower=100  CapacitivePower=100  Pabc=[0 30 25]*1e3/2  QLabc=[0 15 14]*1e3/2  QCabc=[0 0 0]  Pabcp=Pa_836_840/2  QLabcp=Pp_836_840/2  QCabcp=Pn_836_840  Measurements=None  LoadType=constant I
      settings: AttributesFormatString=|
      | P= %<Pabc> W
      | Ql=%<QLabc> var
      | Qc=%<QCabc> var
  836 D-PQ : powerlib/Elements/Three-Phase Series RLC Load  LConnTagsString=A|B|C  Configuration=Delta  NominalVoltage=[  Vabc=[1.017 1.025 1.02]*sqrt(3)*Vnom  Vabcp=V_860_836*Vnom  NominalFrequency=Frequency  UnbalancedPower=on  ActivePower=10e3  InductivePower=100  CapacitivePower=100  Pabc=[0 30 25]*1e3/2  QLabc=[0 15 14]*1e3/2  QCabc=[0 0 0]  Pabcp=Pa_860_836/2  QLabcp=Pp_860_836/2  QCabcp=Pn_860_836  Measurements=None  LoadType=constant PQ
      settings: AttributesFormatString=|
      | P= %<Pabc> W
      | Ql=%<QLabc> var
      | Qc=%<QCabc> var
  836-840 : powerlib/Elements/Distributed Parameters Line  Phases=3  Frequency=Frequency  Resistance=R_301  Inductance=L_301  Capacitance=C_301  Length=860*ft2km  x1=[626.548128535058 24226.3423367686 24183.1524879464;376.991118430775 376.991118430775 376.991118430775;-0.541716681622256 0.18053213741833 1.73938908374105]  x2=[626.508268233823 24225.7298212361 24182.4895385935;376.991118430775 376.991118430775 376.991118430775;-0.541696813328502 0.180530727064737 1.7393967395767]  x3=[0.655281215458781 68.6121500804158 57.1073231593055;376.991118430775 376.991118430775 376.991118430775;-0.438621673700455 0.191066158311745 1.76610834238285]  x4=[0.71924541049129 72.3914292267215 60.2902973268171;376.991118430775 376.991118430775 376.991118430775;-0.636022919480132 0.170191775416098 1.71373896977637]  x5=1.18593158727846e-06  V1=ones(3,3)  V2=ones(3,3)  I1=ones(3,3)  I2=ones(3,3)  nHarmo=1  Measurements=None
  836-862 : powerlib/Elements/Distributed Parameters Line  Phases=3  Frequency=Frequency  Resistance=R_301  Inductance=L_301  Capacitance=C_301  Length=280*ft2km  x1=[626.548213093425 24226.3421736765 24183.1524433828;376.991118430775 376.991118430775 376.991118430775;-0.54141493997098 0.180777872080283 1.73963097269092]  x2=[626.467027740001 24226.21620073 24183.0431247532;376.991118430775 376.991118430775 376.991118430775;-0.540948866788133 0.1807732649742 1.739635331626]  x3=[2.10970006987406 68.8949250513753 58.2612481889625;376.991118430775 376.991118430775 376.991118430775;0.197011730489265 0.173424860836061 1.76410165098693]  x4=[1.43280791034186 72.1631249642583 59.1717145916271;376.991118430775 376.991118430775 376.991118430775;-2.24668211128293 0.187677411406706 1.71542534135381]  x5=3.86117260974383e-07  V1=ones(3,3)  V2=ones(3,3)  I1=ones(3,3)  I2=ones(3,3)  nHarmo=1  Measurements=None
  838 : powerlib/Measurements/Three-Phase V-I Measurement  VoltageMeasurement=phase-to-ground  SetLabelV=on  LabelV=Vabc_838  Vpu=on  VpuLL=off  CurrentMeasurement=yes  SetLabelI=on  LabelI=Iabc_838  Ipu=on  Pbase=base_current  Vbase=Vnom_ph_ph  OutputType=Magnitude-Angle  PhasorSimulation=on  PSBequivalent=0
  838 Y-PQ : powerlib/Elements/Series RLC Load  LConnTagsString=a  RConnTagsString=__new0  NominalVoltage=V_862_838*Vnom  NominalFrequency=Frequency  ActivePower=Pa_862_838/2  InductivePower=Pp_862_838/2  CapacitivePower=Pn_862_838  Setx0=off  InitialVoltage=0  SetiL0=off  InitialCurrent=0  Measurements=None  LoadType=constant PQ
      settings: AttributesFormatString=|
      | P=%<ActivePower> W
      | Ql=%<InductivePower> var
      | Qc=%<CapacitivePower> var
  840 : powerlib/Measurements/Three-Phase V-I Measurement  VoltageMeasurement=phase-to-ground  SetLabelV=on  LabelV=Vabc_840  Vpu=on  VpuLL=off  CurrentMeasurement=yes  SetLabelI=on  LabelI=Iabc_840  Ipu=on  Pbase=base_current  Vbase=Vnom_ph_ph  OutputType=Magnitude-Angle  PhasorSimulation=on  PSBequivalent=0
  840 D-I : powerlib/Elements/Three-Phase Series RLC Load  LConnTagsString=A|B|C  Configuration=Delta  NominalVoltage=[  Vabc=[1.017 1.025 1.02]*sqrt(3)*Vnom  Vabcp=V_836_840*Vnom  NominalFrequency=Frequency  UnbalancedPower=on  ActivePower=10e3  InductivePower=100  CapacitivePower=100  Pabc=[0 30 25]*1e3/2  QLabc=[0 15 14]*1e3/2  QCabc=[0 0 0]  Pabcp=Pa_836_840/2  QLabcp=Pp_836_840/2  QCabcp=Pn_836_840  Measurements=None  LoadType=constant I
      settings: AttributesFormatString=|
      | P= %<Pabc> W
      | Ql=%<QLabc> var
      | Qc=%<QCabc> var
  840 Y-I : powerlib/Elements/Three-Phase Series RLC Load  LConnTagsString=A|B|C  Configuration=Y (grounded)  NominalVoltage=1000  Vabc=V_840*Vnom  Vabcp=[1e3 1e3 1e3]  NominalFrequency=Frequency  UnbalancedPower=on  ActivePower=10e3  InductivePower=100  CapacitivePower=100  Pabc=Pa_840  QLabc=Pp_840  QCabc=Pn_840  Pabcp=[10e3 9e3 11e3]  QLabcp=[100 90 110]  QCabcp=[100 90 110]  Measurements=None  LoadType=constant I
      settings: AttributesFormatString=|
      | P= %<Pabc> W
      | Ql=%<QLabc> var
      | Qc=%<QCabc> var
  842 : powerlib/Measurements/Three-Phase V-I Measurement  VoltageMeasurement=phase-to-ground  SetLabelV=on  LabelV=Vabc_842  Vpu=on  VpuLL=off  CurrentMeasurement=yes  SetLabelI=on  LabelI=Iabc_842  Ipu=on  Pbase=base_current  Vbase=Vnom_ph_ph  OutputType=Magnitude-Angle  PhasorSimulation=on  PSBequivalent=0
  842 Y-PQ : powerlib/Elements/Three-Phase Series RLC Load  LConnTagsString=A|B|C  Configuration=Y (grounded)  NominalVoltage=[  Vabc=V_842_844*Vnom  Vabcp=[1.031 1.029 1.031]*sqrt(3)*Vnom  NominalFrequency=Frequency  UnbalancedPower=on  ActivePower=10e3  InductivePower=100  CapacitivePower=100  Pabc=Pa_842_844/2  QLabc=Pp_842_844/2  QCabc=Pn_842_844  Pabcp=[16 20 110]*1e3/2  QLabcp=[8 10 55]*1e3/2  QCabcp=[0 0 0]  Measurements=None  LoadType=constant PQ
      settings: AttributesFormatString=|
      | P= %<Pabc> W
      | Ql=%<QLabc> var
      | Qc=%<QCabc> var
  842-844 : powerlib/Elements/Distributed Parameters Line  Phases=3  Frequency=Frequency  Resistance=R_301  Inductance=L_301  Capacitance=C_301  Length=1350*ft2km  x1=[629.171950440656 24241.8892384643 24198.3112498873;376.991118430775 376.991118430775 376.991118430775;-0.549953804358248 0.180083878492493 1.738918920697]  x2=[629.708325005518 24243.3215220309 24201.0164820025;376.991118430775 376.991118430775 376.991118430775;-0.550639637411573 0.179001097672016 1.73786454001226]  x3=[1.07877685046548 72.0836129217659 62.1500717840419;376.991118430775 376.991118430775 376.991118430775;-1.36409994251375 -0.617355000150337 0.840866129490908]  x4=[1.0074785983881 104.275282831574 92.432577716875;376.991118430775 376.991118430775 376.991118430775;0.340968856084706 0.696240231440227 2.29146172932197]  x5=1.86163679398363e-06  V1=ones(3,3)  V2=ones(3,3)  I1=ones(3,3)  I2=ones(3,3)  nHarmo=1  Measurements=None
  844 : powerlib/Measurements/Three-Phase V-I Measurement  VoltageMeasurement=phase-to-ground  SetLabelV=on  LabelV=Vabc_844  Vpu=on  VpuLL=off  CurrentMeasurement=yes  SetLabelI=on  LabelI=Iabc_844  Ipu=on  Pbase=base_current  Vbase=Vnom_ph_ph  OutputType=Magnitude-Angle  PhasorSimulation=on  PSBequivalent=0
  844 Y-PQ : powerlib/Elements/Three-Phase Series RLC Load  LConnTagsString=A|B|C  Configuration=Y (grounded)  NominalVoltage=[  Vabc=V_842_844*Vnom  Vabcp=[1.031 1.029 1.031]*sqrt(3)*Vnom  NominalFrequency=Frequency  UnbalancedPower=on  ActivePower=10e3  InductivePower=100  CapacitivePower=100  Pabc=Pa_842_844/2  QLabc=Pp_842_844/2  QCabc=Pn_842_844  Pabcp=[16 20 110]*1e3/2  QLabcp=[8 10 55]*1e3/2  QCabcp=[0 0 0]  Measurements=None  LoadType=constant PQ
      settings: AttributesFormatString=|
      | P= %<Pabc> W
      | Ql=%<QLabc> var
      | Qc=%<QCabc> var
  844 Y-PQ1 : powerlib/Elements/Three-Phase Series RLC Load  LConnTagsString=A|B|C  Configuration=Y (grounded)  NominalVoltage=[  Vabc=V_844_846*Vnom  Vabcp=[1.031 1.029 1.031]*sqrt(3)*Vnom  NominalFrequency=Frequency  UnbalancedPower=on  ActivePower=10e3  InductivePower=100  CapacitivePower=100  Pabc=Pa_844_846/2  QLabc=Pp_844_846/2  QCabc=Pn_844_846  Pabcp=[16 20 110]*1e3/2  QLabcp=[8 10 55]*1e3/2  QCabcp=[0 0 0]  Measurements=None  LoadType=constant PQ
      settings: AttributesFormatString=|
      | P= %<Pabc> W
      | Ql=%<QLabc> var
      | Qc=%<QCabc> var
  844 Y-Z : powerlib/Elements/Three-Phase Series RLC Load  LConnTagsString=A|B|C  Configuration=Y (grounded)  NominalVoltage=[  Vabc=V_844*Vnom  Vabcp=[1.031 1.029 1.031]*sqrt(3)*Vnom  NominalFrequency=Frequency  UnbalancedPower=on  ActivePower=10e3  InductivePower=100  CapacitivePower=100  Pabc=Pa_844  QLabc=Pp_844  QCabc=[0 0 0]  Pabcp=[16 20 110]*1e3/2  QLabcp=[8 10 55]*1e3/2  QCabcp=[0 0 0]  Measurements=Branch voltages and currents  LoadType=constant Z
      settings: AttributesFormatString=|
      | P= %<Pabc> W
      | Ql=%<QLabc> var
      | Qc=%<QCabc> var
  844 Y-Z1 : powerlib/Elements/Three-Phase Series RLC Load  LConnTagsString=A|B|C  Configuration=Y (grounded)  NominalVoltage=[  Vabc="[1  1  1]*Vnom"  Vabcp=[1.031 1.029 1.031]*sqrt(3)*Vnom  NominalFrequency=Frequency  UnbalancedPower=on  ActivePower=10e3  InductivePower=100  CapacitivePower=100  Pabc=[0 0 0]  QLabc=[0 0 0]  QCabc=Pn_844  Pabcp=[16 20 110]*1e3/2  QLabcp=[8 10 55]*1e3/2  QCabcp=[0 0 0]  Measurements=None  LoadType=constant Z
      settings: AttributesFormatString=|
      | P= %<Pabc> W
      | Ql=%<QLabc> var
      | Qc=%<QCabc> var
  844-846 : powerlib/Elements/Distributed Parameters Line  Phases=3  Frequency=Frequency  Resistance=R_301  Inductance=L_301  Capacitance=C_301  Length=3640*ft2km  x1=[629.708325005518 24243.3215220309 24201.0164820025;376.991118430775 376.991118430775 376.991118430775;-0.551830132989279 0.178030861198964 1.73690951848382]  x2=[631.86711889889 24265.7665577817 24227.4499677873;376.991118430775 376.991118430775 376.991118430775;-0.554038378829758 0.17546185324734 1.73445292523355]  x3=[1.38248672481002 83.876052108821 73.6801064917891;376.991118430775 376.991118430775 376.991118430775;-1.43888002284194 -0.483913792577468 1.00425667990267]  x4=[1.18109788943462 90.6205884115728 79.4839195535622;376.991118430775 376.991118430775 376.991118430775;0.579553931024776 0.779322474010274 2.40192444146512]  x5=5.01952439266698e-06  V1=ones(3,3)  V2=ones(3,3)  I1=ones(3,3)  I2=ones(3,3)  nHarmo=1  Measurements=None
  846 : powerlib/Measurements/Three-Phase V-I Measurement  VoltageMeasurement=phase-to-ground  SetLabelV=on  LabelV=Vabc_846  Vpu=on  VpuLL=off  CurrentMeasurement=yes  SetLabelI=on  LabelI=Iabc_846  Ipu=on  Pbase=base_current  Vbase=Vnom_ph_ph  OutputType=Magnitude-Angle  PhasorSimulation=on  PSBequivalent=0
  846 Y-PQ : powerlib/Elements/Three-Phase Series RLC Load  LConnTagsString=A|B|C  Configuration=Y (grounded)  NominalVoltage=[  Vabc=V_844_846*Vnom  Vabcp=[1.031 1.029 1.031]*sqrt(3)*Vnom  NominalFrequency=Frequency  UnbalancedPower=on  ActivePower=10e3  InductivePower=100  CapacitivePower=100  Pabc=Pa_844_846/2  QLabc=Pp_844_846/2  QCabc=Pn_844_846  Pabcp=[16 20 110]*1e3/2  QLabcp=[8 10 55]*1e3/2  QCabcp=[0 0 0]  Measurements=None  LoadType=constant PQ
      settings: AttributesFormatString=|
      | P= %<Pabc> W
      | Ql=%<QLabc> var
      | Qc=%<QCabc> var
  846 Y-PQ1 : powerlib/Elements/Three-Phase Series RLC Load  LConnTagsString=A|B|C  Configuration=Y (grounded)  NominalVoltage=[  Vabc=V_846_848*Vnom  Vabcp=[1.031 1.029 1.031]*sqrt(3)*Vnom  NominalFrequency=Frequency  UnbalancedPower=on  ActivePower=10e3  InductivePower=100  CapacitivePower=100  Pabc=Pa_846_848/2  QLabc=Pp_846_848/2  QCabc=Pn_846_848  Pabcp=[16 20 110]*1e3/2  QLabcp=[8 10 55]*1e3/2  QCabcp=[0 0 0]  Measurements=None  LoadType=constant PQ
      settings: AttributesFormatString=|
      | P= %<Pabc> W
      | Ql=%<QLabc> var
      | Qc=%<QCabc> var
  846-848 : powerlib/Elements/Distributed Parameters Line  Phases=3  Frequency=Frequency  Resistance=R_301  Inductance=L_301  Capacitance=C_301  Length=530*ft2km  x1=[631.86711889889 24265.7665577817 24227.4499677873;376.991118430775 376.991118430775 376.991118430775;-0.552421592259161 0.176779510640873 1.73574991953636]  x2=[632.12872379164 24269.2555615764 24231.6431399049;376.991118430775 376.991118430775 376.991118430775;-0.553402316056239 0.17641216620611 1.735387294071]  x3=[1.7863854336738 85.073047395481 75.7576723040171;376.991118430775 376.991118430775 376.991118430775;-2.18901783147898 -0.470582436649014 1.00197258091048]  x4=[2.32734637250788 89.5372457044052 79.5840804185877;376.991118430775 376.991118430775 376.991118430775;0.319442567736115 0.786390173453038 2.42641516474851]  x5=7.30864815415796e-07  V1=ones(3,3)  V2=ones(3,3)  I1=ones(3,3)  I2=ones(3,3)  nHarmo=1  Measurements=None
  848 : powerlib/Measurements/Three-Phase V-I Measurement  VoltageMeasurement=phase-to-ground  SetLabelV=on  LabelV=Vabc_848  Vpu=on  VpuLL=off  CurrentMeasurement=yes  SetLabelI=on  LabelI=Iabc_848  Ipu=on  Pbase=base_current  Vbase=Vnom_ph_ph  OutputType=Magnitude-Angle  PhasorSimulation=on  PSBequivalent=0
  848 D-PQ : powerlib/Elements/Three-Phase Series RLC Load  LConnTagsString=A|B|C  Configuration=Delta  NominalVoltage=1000  Vabc=[1e3 1e3 1e3]  Vabcp=V_848*Vnom  NominalFrequency=Frequency  UnbalancedPower=on  ActivePower=[20 20 20]*1e3  InductivePower=[20 20 20]*1e3  CapacitivePower=100  Pabc=[10e3 9e3 11e3]  QLabc=[100 90 110]  QCabc=[100 90 110]  Pabcp=Pa_848  QLabcp=Pp_848  QCabcp=[0 0 0]  Measurements=Branch voltages and currents  LoadType=constant PQ
      settings: AttributesFormatString=|
      | P= %<Pabc> W
      | Ql=%<QLabc> var
      | Qc=%<QCabc> var
  848 D-Z : powerlib/Elements/Three-Phase Series RLC Load  LConnTagsString=A|B|C  Configuration=Delta  NominalVoltage=1000  Vabc=[1e3 1e3 1e3]  Vabcp="[1  1  1]*Vnom"  NominalFrequency=Frequency  UnbalancedPower=on  ActivePower=[20 20 20]*1e3  InductivePower=[20 20 20]*1e3  CapacitivePower=100  Pabc=[10e3 9e3 11e3]  QLabc=[100 90 110]  QCabc=[100 90 110]  Pabcp=[0 0 0]  QLabcp=[0 0 0]  QCabcp=Pn_848  Measurements=None  LoadType=constant Z
      settings: AttributesFormatString=|
      | P= %<Pabc> W
      | Ql=%<QLabc> var
      | Qc=%<QCabc> var
  848 Y-PQ : powerlib/Elements/Three-Phase Series RLC Load  LConnTagsString=A|B|C  Configuration=Y (grounded)  NominalVoltage=[  Vabc=V_846_848*Vnom  Vabcp=[1.031 1.029 1.031]*sqrt(3)*Vnom  NominalFrequency=Frequency  UnbalancedPower=on  ActivePower=10e3  InductivePower=100  CapacitivePower=100  Pabc=Pa_846_848/2  QLabc=Pp_846_848/2  QCabc=Pn_846_848  Pabcp=[16 20 110]*1e3/2  QLabcp=[8 10 55]*1e3/2  QCabcp=[0 0 0]  Measurements=None  LoadType=constant PQ
      settings: AttributesFormatString=|
      | P= %<Pabc> W
      | Ql=%<QLabc> var
      | Qc=%<QCabc> var
  850 : powerlib/Measurements/Three-Phase V-I Measurement  VoltageMeasurement=phase-to-ground  SetLabelV=on  LabelV=Vabc_850  Vpu=on  VpuLL=off  CurrentMeasurement=yes  SetLabelI=on  LabelI=Iabc_850  Ipu=on  Pbase=base_current  Vbase=Vnom_ph_ph  OutputType=Magnitude-Angle  PhasorSimulation=on  PSBequivalent=0
  850-816 : powerlib/Elements/Distributed Parameters Line  Phases=3  Frequency=Frequency  Resistance=R_301  Inductance=L_301  Capacitance=C_301  Length=310*ft2km  x1=[749.971237422085 25228.9617411345 25142.3976995942;376.991118430775 376.991118430775 376.991118430775;-0.624316781537292 0.23746636263491 1.80399152362199]  x2=[749.254552412162 25224.3500731886 25137.8871613909;376.991118430775 376.991118430775 376.991118430775;-0.623592971369802 0.237246574337769 1.8037518217745]  x3=[4.46412545478375 31.9558028962219 28.1820456886809;376.991118430775 376.991118430775 376.991118430775;0.861899197520254 -0.884669954931422 0.236083292401272]  x4=[4.62267432898314 136.09008098403 125.16934102869;376.991118430775 376.991118430775 376.991118430775;-1.9191021475991 0.450457543166538 2.03090431600836]  x5=4.27486967507352e-07  V1=ones(3,3)  V2=ones(3,3)  I1=ones(3,3)  I2=ones(3,3)  nHarmo=1  Measurements=None
  852 : powerlib/Measurements/Three-Phase V-I Measurement  VoltageMeasurement=phase-to-ground  SetLabelV=on  LabelV=Vabc_852  Vpu=on  VpuLL=off  CurrentMeasurement=yes  SetLabelI=on  LabelI=Iabc_852  Ipu=on  Pbase=base_current  Vbase=Vnom_ph_ph  OutputType=Magnitude-Angle  PhasorSimulation=on  PSBequivalent=0
  852-832 : powerlib/Elements/Distributed Parameters Line  Phases=3  Frequency=Frequency  Resistance=R_301  Inductance=L_301  Capacitance=C_301  Length=10*ft2km  x1=[636.242340422448 24296.5745757526 24244.2562748666;376.991118430775 376.991118430775 376.991118430775;-0.55792766668964 0.188835125792642 1.74852529686162]  x2=[636.228321854336 24296.4474030039 24244.1353008069;376.991118430775 376.991118430775 376.991118430775;-0.557919216213416 0.18882795778521 1.74851710931291]  x3=[2.15556641718706 34.739479075958 32.5822545216707;376.991118430775 376.991118430775 376.991118430775;1.0893510507275 -0.86064554442103 0.280316798448705]  x4=[2.65231633685663 127.790388516075 118.879815111722;376.991118430775 376.991118430775 376.991118430775;-1.5026499216019 0.426804915402872 2.02465101063265]  x5=1.37899021776565e-08  V1=ones(3,3)  V2=ones(3,3)  I1=ones(3,3)  I2=ones(3,3)  nHarmo=1  Measurements=None
  854 : powerlib/Measurements/Three-Phase V-I Measurement  VoltageMeasurement=phase-to-ground  SetLabelV=on  LabelV=Vabc_854  Vpu=on  VpuLL=off  CurrentMeasurement=yes  SetLabelI=on  LabelI=Iabc_854  Ipu=on  Pbase=base_current  Vbase=Vnom_ph_ph  OutputType=Magnitude-Angle  PhasorSimulation=on  PSBequivalent=0
  854 Y-PQ : powerlib/Elements/Series RLC Load  LConnTagsString=a  RConnTagsString=__new0  NominalVoltage=V_854_856*Vnom  NominalFrequency=Frequency  ActivePower=Pa_854_856/2  InductivePower=Pp_854_856/2  CapacitivePower=Pn_854_856  Setx0=off  InitialVoltage=0  SetiL0=off  InitialCurrent=0  Measurements=None  LoadType=constant PQ
      settings: AttributesFormatString=|
      | P=%<ActivePower> W
      | Ql=%<InductivePower> var
      | Qc=%<CapacitivePower> var
  854-852 : powerlib/Elements/Distributed Parameters Line  Phases=3  Frequency=Frequency  Resistance=R_301  Inductance=L_301  Capacitance=C_301  Length=36830*ft2km  x1=[688.035917811594 24770.3844862052 24697.8456577878;376.991118430775 376.991118430775 376.991118430775;-0.60568888849568 0.199396157636819 1.76298984479971]  x2=[636.242340422448 24296.5745757526 24244.2562748666;376.991118430775 376.991118430775 376.991118430775;-0.577069172004551 0.173235079094923 1.73316988521231]  x3=[2.09831784614322 33.8897362974249 31.3519440680455;376.991118430775 376.991118430775 376.991118430775;1.04664370528229 -0.846291352664001 0.288545462694233]  x4=[2.62716428361621 125.043088148097 116.807618884584;376.991118430775 376.991118430775 376.991118430775;-1.5227235695919 0.412325115292594 2.01025698192622]  x5=5.0788209720309e-05  V1=ones(3,3)  V2=ones(3,3)  I1=ones(3,3)  I2=ones(3,3)  nHarmo=1  Measurements=None
  854-856 : powerlib/Elements/Distributed Parameters Line  Phases=1  Frequency=Frequency  Resistance=R_303(2,2)  Inductance=L_303(2,2)  Capacitance=C_303(2,2)  Length=23330*ft2km  x1=[20201.0846397519;376.991118430775;-2.20057250543352]  x2=[20199.2504210947;376.991118430775;-2.20069164551243]  x3=[33.3472579130479;376.991118430775;-2.2088512995778]  x4=[33.731673397818;376.991118430775;-2.2035705641835]  x5=2.9363349960162e-05  V1=ones(3,3)  V2=ones(3,3)  I1=ones(3,3)  I2=ones(3,3)  nHarmo=1  Measurements=None
  856 : powerlib/Measurements/Three-Phase V-I Measurement  VoltageMeasurement=phase-to-ground  SetLabelV=on  LabelV=Vabc_856  Vpu=on  VpuLL=off  CurrentMeasurement=yes  SetLabelI=on  LabelI=Iabc_856  Ipu=on  Pbase=base_current  Vbase=Vnom_ph_ph  OutputType=Magnitude-Angle  PhasorSimulation=on  PSBequivalent=0
  856 Y-PQ : powerlib/Elements/Series RLC Load  LConnTagsString=a  RConnTagsString=__new0  NominalVoltage=V_854_856*Vnom  NominalFrequency=Frequency  ActivePower=Pa_854_856/2  InductivePower=Pp_854_856/2  CapacitivePower=Pn_854_856  Setx0=off  InitialVoltage=0  SetiL0=off  InitialCurrent=0  Measurements=None  LoadType=constant PQ
      settings: AttributesFormatString=|
      | P=%<ActivePower> W
      | Ql=%<InductivePower> var
      | Qc=%<CapacitivePower> var
  858 : powerlib/Measurements/Three-Phase V-I Measurement  VoltageMeasurement=phase-to-ground  SetLabelV=on  LabelV=Vabc_858  Vpu=on  VpuLL=off  CurrentMeasurement=yes  SetLabelI=on  LabelI=Iabc_858  Ipu=on  Pbase=base_current  Vbase=Vnom_ph_ph  OutputType=Magnitude-Angle  PhasorSimulation=on  PSBequivalent=0
  858 D-PQ : powerlib/Elements/Three-Phase Series RLC Load  LConnTagsString=A|B|C  Configuration=Delta  NominalVoltage=[  Vabc=[1.017 1.025 1.02]*sqrt(3)*Vnom  Vabcp=V_858_834*Vnom  NominalFrequency=Frequency  UnbalancedPower=on  ActivePower=10e3  InductivePower=100  CapacitivePower=100  Pabc=[0 30 25]*1e3/2  QLabc=[0 15 14]*1e3/2  QCabc=[0 0 0]  Pabcp=Pa_858_834/2  QLabcp=Pp_858_834/2  QCabcp=Pn_858_834  Measurements=None  LoadType=constant PQ
      settings: AttributesFormatString=|
      | P= %<Pabc> W
      | Ql=%<QLabc> var
      | Qc=%<QCabc> var
  858 D-Z : powerlib/Elements/Three-Phase Series RLC Load  LConnTagsString=A|B|C  Configuration=Delta  NominalVoltage=[  Vabc=[1.017 1.025 1.02]*sqrt(3)*Vnom  Vabcp=V_832_858*Vnom  NominalFrequency=Frequency  UnbalancedPower=on  ActivePower=10e3  InductivePower=100  CapacitivePower=100  Pabc=[0 30 25]*1e3/2  QLabc=[0 15 14]*1e3/2  QCabc=[0 0 0]  Pabcp=Pa_832_858/2  QLabcp=Pp_832_858/2  QCabcp=Pn_832_858  Measurements=None  LoadType=constant Z
      settings: AttributesFormatString=|
      | P= %<Pabc> W
      | Ql=%<QLabc> var
      | Qc=%<QCabc> var
  858 Y-PQ : powerlib/Elements/Series RLC Load  LConnTagsString=a  RConnTagsString=__new0  NominalVoltage=1.034*Vnom  NominalFrequency=Frequency  ActivePower=Pa_858_864/2  InductivePower=Pp_858_864/2  CapacitivePower=Pn_858_864  Setx0=off  InitialVoltage=0  SetiL0=off  InitialCurrent=0  Measurements=None  LoadType=constant PQ
      settings: AttributesFormatString=|
      | P=%<ActivePower> W
      | Ql=%<InductivePower> var
      | Qc=%<CapacitivePower> var
  858-834 : powerlib/Elements/Distributed Parameters Line  Phases=3  Frequency=Frequency  Resistance=R_301  Inductance=L_301  Capacitance=C_301  Length=5830*ft2km  x1=[632.750499487762 24270.3723308237 24221.7201740198;376.991118430775 376.991118430775 376.991118430775;-0.557165864707982 0.182735174887884 1.74205580142964]  x2=[629.097777973359 24241.6292315875 24197.757448572;376.991118430775 376.991118430775 376.991118430775;-0.552084232926923 0.178410153067586 1.73726997564012]  x3=[1.43839890045908 54.6185367237257 48.3845616376066;376.991118430775 376.991118430775 376.991118430775;0.542761792674936 -0.657980680962952 0.654190081455323]  x4=[1.47020503952244 111.742295659643 103.752575406271;376.991118430775 376.991118430775 376.991118430775;-1.61428588828557 0.550927799470993 2.16334644277604]  x5=8.03951296957376e-06  V1=ones(3,3)  V2=ones(3,3)  I1=ones(3,3)  I2=ones(3,3)  nHarmo=1  Measurements=None
  858-864 : powerlib/Elements/Distributed Parameters Line  Phases=1  Frequency=Frequency  Resistance=R_302(1,1)  Inductance=L_302(1,1)  Capacitance=C_302(1,1)  Length=1620*ft2km  x1=[19660.2431210964;376.991118430775;-0.102752214493179]  x2=[19660.1522284335;376.991118430775;-0.102752890298995]  x3=[33.0317748732336;376.991118430775;-0.102177388445182]  x4=[33.2094673366351;376.991118430775;-0.10409152483685]  x5=2.03894671819385e-06  V1=ones(3,3)  V2=ones(3,3)  I1=ones(3,3)  I2=ones(3,3)  nHarmo=1  Measurements=None
  860 : powerlib/Measurements/Three-Phase V-I Measurement  VoltageMeasurement=phase-to-ground  SetLabelV=on  LabelV=Vabc_860  Vpu=on  VpuLL=off  CurrentMeasurement=yes  SetLabelI=on  LabelI=Iabc_860  Ipu=on  Pbase=base_current  Vbase=Vnom_ph_ph  OutputType=Magnitude-Angle  PhasorSimulation=on  PSBequivalent=0
  860 D-PQ : powerlib/Elements/Three-Phase Series RLC Load  LConnTagsString=A|B|C  Configuration=Delta  NominalVoltage=[  Vabc=[1.017 1.025 1.02]*sqrt(3)*Vnom  Vabcp=V_860_836*Vnom  NominalFrequency=Frequency  UnbalancedPower=on  ActivePower=10e3  InductivePower=100  CapacitivePower=100  Pabc=[0 30 25]*1e3/2  QLabc=[0 15 14]*1e3/2  QCabc=[0 0 0]  Pabcp=Pa_860_836/2  QLabcp=Pp_860_836/2  QCabcp=Pn_860_836  Measurements=None  LoadType=constant PQ
      settings: AttributesFormatString=|
      | P= %<Pabc> W
      | Ql=%<QLabc> var
      | Qc=%<QCabc> var
  860 D-Z : powerlib/Elements/Three-Phase Series RLC Load  LConnTagsString=A|B|C  Configuration=Delta  NominalVoltage=[  Vabc=[1.017 1.025 1.02]*sqrt(3)*Vnom  Vabcp=V_834_860*Vnom  NominalFrequency=Frequency  UnbalancedPower=on  ActivePower=10e3  InductivePower=100  CapacitivePower=100  Pabc=[0 30 25]*1e3/2  QLabc=[0 15 14]*1e3/2  QCabc=[0 0 0]  Pabcp=Pa_834_860/2  QLabcp=Pp_834_860/2  QCabcp=Pn_834_860  Measurements=None  LoadType=constant Z
      settings: AttributesFormatString=|
      | P= %<Pabc> W
      | Ql=%<QLabc> var
      | Qc=%<QCabc> var
  860 Y-PQ : powerlib/Elements/Three-Phase Series RLC Load  LConnTagsString=A|B|C  Configuration=Y (grounded)  NominalVoltage=[  Vabc=V_860*Vnom  Vabcp=[1.031 1.029 1.031]*sqrt(3)*Vnom  NominalFrequency=Frequency  UnbalancedPower=on  ActivePower=10e3  InductivePower=100  CapacitivePower=100  Pabc=Pa_860  QLabc=Pp_860  QCabc=Pn_860  Pabcp=[16 20 110]*1e3/2  QLabcp=[8 10 55]*1e3/2  QCabcp=[0 0 0]  Measurements=None  LoadType=constant PQ
      settings: AttributesFormatString=|
      | P= %<Pabc> W
      | Ql=%<QLabc> var
      | Qc=%<QCabc> var
  860-836 : powerlib/Elements/Distributed Parameters Line  Phases=3  Frequency=Frequency  Resistance=R_301  Inductance=L_301  Capacitance=C_301  Length=2680*ft2km  x1=[627.6711248122 24232.0625215145 24188.4434896558;376.991118430775 376.991118430775 376.991118430775;-0.547167652411273 0.179804635279464 1.73856940386009]  x2=[626.548128535058 24226.3423367686 24183.1524879464;376.991118430775 376.991118430775 376.991118430775;-0.542662839679647 0.179761032448481 1.73863007099793]  x3=[2.13280537728672 64.4579886569561 54.688014128491;376.991118430775 376.991118430775 376.991118430775;0.285769132829028 0.202317755440231 1.80974788968011]  x4=[1.57736256598051 76.4088808390813 62.8230269778878;376.991118430775 376.991118430775 376.991118430775;-2.16015641211496 0.159725710407411 1.67563175252492]  x5=3.69569378361195e-06  V1=ones(3,3)  V2=ones(3,3)  I1=ones(3,3)  I2=ones(3,3)  nHarmo=1  Measurements=None
  862 : powerlib/Measurements/Three-Phase V-I Measurement  VoltageMeasurement=phase-to-ground  SetLabelV=on  LabelV=Vabc_862  Vpu=on  VpuLL=off  CurrentMeasurement=yes  SetLabelI=on  LabelI=Iabc_862  Ipu=on  Pbase=base_current  Vbase=Vnom_ph_ph  OutputType=Magnitude-Angle  PhasorSimulation=on  PSBequivalent=0
  862 Y-PQ : powerlib/Elements/Series RLC Load  LConnTagsString=a  RConnTagsString=__new0  NominalVoltage=V_862_838*Vnom  NominalFrequency=Frequency  ActivePower=Pa_862_838/2  InductivePower=Pp_862_838/2  CapacitivePower=Pn_862_838  Setx0=off  InitialVoltage=0  SetiL0=off  InitialCurrent=0  Measurements=None  LoadType=constant PQ
      settings: AttributesFormatString=|
      | P=%<ActivePower> W
      | Ql=%<InductivePower> var
      | Qc=%<CapacitivePower> var
  862-838 : powerlib/Elements/Distributed Parameters Line  Phases=1  Frequency=Frequency  Resistance=R_304(2,2)  Inductance=L_304(2,2)  Capacitance=C_304(2,2)  Length=4860*ft2km  x1=[19781.4619046394;376.991118430775;-2.22886316995273]  x2=[19778.4480104482;376.991118430775;-2.22889382670031]  x3=[33.3230979295555;376.991118430775;-2.2122849931945]  x4=[35.8455876108611;376.991118430775;-2.24651747408965]  x5=6.08033278760362e-06  V1=ones(3,3)  V2=ones(3,3)  I1=ones(3,3)  I2=ones(3,3)  nHarmo=1  Measurements=None
  864 : powerlib/Measurements/Three-Phase V-I Measurement  VoltageMeasurement=phase-to-ground  SetLabelV=on  LabelV=Vabc_864  Vpu=on  VpuLL=off  CurrentMeasurement=yes  SetLabelI=on  LabelI=Iabc_864  Ipu=on  Pbase=base_current  Vbase=Vnom_ph_ph  OutputType=Magnitude-Angle  PhasorSimulation=on  PSBequivalent=0
  864 Y-PQ : powerlib/Elements/Series RLC Load  LConnTagsString=a  RConnTagsString=__new0  NominalVoltage=1.034*Vnom  NominalFrequency=Frequency  ActivePower=2e3/2  InductivePower=1e3/2  CapacitivePower=0  Setx0=off  InitialVoltage=0  SetiL0=off  InitialCurrent=0  Measurements=None  LoadType=constant PQ
      settings: AttributesFormatString=|
      | P=%<ActivePower> W
      | Ql=%<InductivePower> var
      | Qc=%<CapacitivePower> var
  888 : powerlib/Measurements/Three-Phase V-I Measurement  VoltageMeasurement=phase-to-ground  SetLabelV=on  LabelV=Vabc_888  Vpu=on  VpuLL=off  CurrentMeasurement=yes  SetLabelI=on  LabelI=Iabc_888  Ipu=on  Pbase=base_current  Vbase=Vnom1_ph_ph  OutputType=Magnitude-Angle  PhasorSimulation=on  PSBequivalent=0
  888-890 : powerlib/Elements/Distributed Parameters Line  Phases=3  Frequency=Frequency  Resistance=R_300  Inductance=L_300  Capacitance=C_300  Length=10560*ft2km  x1=[255.205386436858 3904.75927901987 3893.90479851016;376.991118430775 376.991118430775 376.991118430775;1.80377872906611 0.156810924017685 1.71910118809817]  x2=[268.899263774576 3573.45761323568 3550.76473817171;376.991118430775 376.991118430775 376.991118430775;1.86877552441132 0.145320105791603 1.69990430632381]  x3=[4.28048219205887 112.802827224234 114.061030288051;376.991118430775 376.991118430775 376.991118430775;1.79645363487912 2.7782797794061 -1.9451709848619]  x4=[3.6487688553485 132.67992857686 130.485385979101;376.991118430775 376.991118430775 376.991118430775;-1.35172186318473 -0.280867772943754 1.26574961384332]  x5=1.41710191462344e-05  V1=ones(3,3)  V2=ones(3,3)  I1=ones(3,3)  I2=ones(3,3)  nHarmo=1  Measurements=None
  890 : powerlib/Measurements/Three-Phase V-I Measurement  VoltageMeasurement=phase-to-ground  SetLabelV=on  LabelV=Vabc_890  Vpu=on  VpuLL=off  CurrentMeasurement=yes  SetLabelI=on  LabelI=Iabc_890  Ipu=on  Pbase=base_current  Vbase=Vnom1_ph_ph  OutputType=Magnitude-Angle  PhasorSimulation=on  PSBequivalent=0
  890 D-I : powerlib/Elements/Three-Phase Series RLC Load  LConnTagsString=A|B|C  Configuration=Delta  NominalVoltage=1000  Vabc=[1e3 1e3 1e3]  Vabcp=V_890*Vnom1  NominalFrequency=Frequency  UnbalancedPower=on  ActivePower=10e3  InductivePower=100  CapacitivePower=100  Pabc=[10e3 9e3 11e3]  QLabc=[100 90 110]  QCabc=[100 90 110]  Pabcp=Pa_890  QLabcp=Pp_890  QCabcp=Pn_890  Measurements=None  LoadType=constant I
  Breaker818-820 : powerlib/Elements/Breaker  InitialState=0  SwitchingTimes="[1/60  5/60]"  External=on  BreakerResistance=0.0001  SnubberResistance=inf  SnubberCapacitance=0  Measurements=None  MoreParameters=on  NoBreakLoop=off
  Breaker832-858 : powerlib/Elements/Three-Phase Breaker  InitialState=closed  SwitchA=on  SwitchB=on  SwitchC=on  SwitchTimes=[0.5 ]  External=on  BreakerResistance=0.0001  SnubberResistance=inf  SnubberCapacitance=0  Measurements=None
  Breaker834-842 : powerlib/Elements/Three-Phase Breaker  InitialState=closed  SwitchA=on  SwitchB=on  SwitchC=on  SwitchTimes=[0.5 ]  External=on  BreakerResistance=0.0001  SnubberResistance=inf  SnubberCapacitance=0  Measurements=None
  Breaker836-862 : powerlib/Elements/Three-Phase Breaker  InitialState=closed  SwitchA=on  SwitchB=on  SwitchC=on  SwitchTimes=[0.5 ]  External=on  BreakerResistance=0.0001  SnubberResistance=inf  SnubberCapacitance=0  Measurements=None
  Breaker850-816 : powerlib/Elements/Three-Phase Breaker  InitialState=closed  SwitchA=on  SwitchB=on  SwitchC=on  SwitchTimes=[0.5 ]  External=on  BreakerResistance=0.0001  SnubberResistance=inf  SnubberCapacitance=0  Measurements=None
  Constant1 : Constant  Value=SW850_816
  Constant2 : Constant  Value=SW818_820
  Constant3 : Constant  Value=SW832_858
  Constant4 : Constant  Value=SW834_842
  Constant5 : Constant  Value=SW836_862
  Ground{,1..21} (22 alike) : powerlib/Elements/Ground  LConnTagsString=a
  Load Flow Bus : powerlib/Measurements/Load Flow Bus  LConnTagsString=a|b|c  RConnTagsString=a|b|c  Phases=ABC  Connectors=on both sides  ID=800  Vbase=Vnom  Vref="[1.05  1.05  1.05]"  Vangle="[0  -120  120]"  VLF=1  VLFb=1  VLFc=1  angleLF=0  angleLFb=0  angleLFc=0
      settings: AttributesFormatString=%<ID>
  Load Flow Bus1 : powerlib/Measurements/Load Flow Bus  LConnTagsString=a|b|c  RConnTagsString=a|b|c  Phases=ABC  Connectors=on both sides  ID=802  Vbase=Vnom  Vref=[1.0475 1.0484 1.0484]  Vangle=[-0.05 -120.07 119.95]  VLF=1  VLFb=1  VLFc=1  angleLF=0  angleLFb=0  angleLFc=0
      settings: AttributesFormatString=%<ID>
  Load Flow Bus10 : powerlib/Measurements/Load Flow Bus  LConnTagsString=a  Phases=B  Connectors=on one side  ID=826  Vbase=Vnom  Vref=1.0156  Vangle=-122.94  VLF=1  VLFb=1  VLFc=1  angleLF=0  angleLFb=0  angleLFc=0
      settings: AttributesFormatString=%<ID>
  Load Flow Bus11 : powerlib/Measurements/Load Flow Bus  LConnTagsString=a  RConnTagsString=a  Phases=A  Connectors=on both sides  ID=818  Vbase=Vnom  Vref=1.0163  Vangle=-2.27  VLF=1  VLFb=1  VLFc=1  angleLF=0  angleLFb=0  angleLFc=0
      settings: AttributesFormatString=%<ID>
  Load Flow Bus12 : powerlib/Measurements/Load Flow Bus  LConnTagsString=a  RConnTagsString=a  Phases=A  Connectors=on both sides  ID=820  Vbase=Vnom  Vref=0.9926  Vangle=-2.32  VLF=1  VLFb=1  VLFc=1  angleLF=0  angleLFb=0  angleLFc=0
      settings: AttributesFormatString=%<ID>
  Load Flow Bus13 : powerlib/Measurements/Load Flow Bus  LConnTagsString=a  Phases=A  Connectors=on one side  ID=822  Vbase=Vnom  Vref=0.9895  Vangle=-2.33  VLF=1  VLFb=1  VLFc=1  angleLF=0  angleLFb=0  angleLFc=0
      settings: AttributesFormatString=%<ID>
  Load Flow Bus14 : powerlib/Measurements/Load Flow Bus  LConnTagsString=a|b|c  RConnTagsString=a|b|c  Phases=ABC  Connectors=on both sides  ID=828  Vbase=Vnom  Vref=[1.0074 1.0151 1.0109]  Vangle=[-2.38 -122.95 117.75]  VLF=1  VLFb=1  VLFc=1  angleLF=0  angleLFb=0  angleLFc=0
      settings: AttributesFormatString=%<ID>
  Load Flow Bus15 : powerlib/Measurements/Load Flow Bus  LConnTagsString=a|b|c  RConnTagsString=a|b|c  Phases=ABC  Connectors=on both sides  ID=830  Vbase=Vnom  Vref=[0.9894 0.9982 0.9938]  Vangle=[-2.63 -123.39 117.25]  VLF=1  VLFb=1  VLFc=1  angleLF=0  angleLFb=0  angleLFc=0
      settings: AttributesFormatString=%<ID>
  Load Flow Bus16 : powerlib/Measurements/Load Flow Bus  LConnTagsString=a|b|c  RConnTagsString=a|b|c  Phases=ABC  Connectors=on both sides  ID=854  Vbase=Vnom  Vref=[0.989 0.9978 0.9934]  Vangle=[-2.64 -123.4 117.24]  VLF=1  VLFb=1  VLFc=1  angleLF=0  angleLFb=0  angleLFc=0
      settings: AttributesFormatString=%<ID>
  Load Flow Bus17 : powerlib/Measurements/Load Flow Bus  LConnTagsString=a  Phases=B  Connectors=on one side  ID=856  Vbase=Vnom  Vref=0.9977  Vangle=-123.41  VLF=1  VLFb=1  VLFc=1  angleLF=0  angleLFb=0  angleLFc=0
      settings: AttributesFormatString=%<ID>
  Load Flow Bus18 : powerlib/Measurements/Load Flow Bus  LConnTagsString=a|b|c  RConnTagsString=a|b|c  Phases=ABC  Connectors=on both sides  ID=852  Vbase=Vnom  Vref=[0.9581 0.968 0.9637]  Vangle=[-3.11 -124.18 116.33]  VLF=1  VLFb=1  VLFc=1  angleLF=0  angleLFb=0  angleLFc=0
      settings: AttributesFormatString=%<ID>
  Load Flow Bus19 : powerlib/Measurements/Load Flow Bus  LConnTagsString=a|b|c  RConnTagsString=a|b|c  Phases=ABC  Connectors=on both sides  ID=832  Vbase=Vnom  Vref=[1.0359 1.0345 1.036]  Vangle=[-3.11 -124.18 116.33]  VLF=1  VLFb=1  VLFc=1  angleLF=0  angleLFb=0  angleLFc=0
      settings: AttributesFormatString=%<ID>
  Load Flow Bus2 : powerlib/Measurements/Load Flow Bus  LConnTagsString=a|b|c  RConnTagsString=a|b|c  Phases=ABC  Connectors=on both sides  ID=806  Vbase=Vnom  Vref=[1.0457 1.0474 1.0474]  Vangle=[-0.08 -120.11 119.92]  VLF=1  VLFb=1  VLFc=1  angleLF=0  angleLFb=0  angleLFc=0
      settings: AttributesFormatString=%<ID>
  Load Flow Bus20 : powerlib/Measurements/Load Flow Bus  LConnTagsString=a|b|c  RConnTagsString=a|b|c  Phases=ABC  Connectors=on both sides  ID=888  Vbase=Vnom1  Vref=[0.9996 0.9983 1]  Vangle=[-4.64 -125.73 114.82]  VLF=1  VLFb=1  VLFc=1  angleLF=0  angleLFb=0  angleLFc=0
      settings: AttributesFormatString=%<ID>
  Load Flow Bus21 : powerlib/Measurements/Load Flow Bus  LConnTagsString=a|b|c  RConnTagsString=a|b|c  Phases=ABC  Connectors=on both sides  ID=890  Vbase=Vnom1  Vref=[0.9167 0.9235 0.9177]  Vangle=[-5.19 -126.78 113.98]  VLF=1  VLFb=1  VLFc=1  angleLF=0  angleLFb=0  angleLFc=0
      settings: AttributesFormatString=%<ID>
  Load Flow Bus22 : powerlib/Measurements/Load Flow Bus  LConnTagsString=a|b|c  RConnTagsString=a|b|c  Phases=ABC  Connectors=on both sides  ID=858  Vbase=Vnom  Vref=[1.0336 1.0322 1.0338]  Vangle=[-3.17 -124.28 116.22]  VLF=1  VLFb=1  VLFc=1  angleLF=0  angleLFb=0  angleLFc=0
      settings: AttributesFormatString=%<ID>
  Load Flow Bus23 : powerlib/Measurements/Load Flow Bus  LConnTagsString=a  Phases=A  Connectors=on one side  ID=864  Vbase=Vnom  Vref=1.0336  Vangle=-3.17  VLF=1  VLFb=1  VLFc=1  angleLF=0  angleLFb=0  angleLFc=0
      settings: AttributesFormatString=%<ID>
  Load Flow Bus24 : powerlib/Measurements/Load Flow Bus  LConnTagsString=a|b|c  RConnTagsString=a|b|c  Phases=ABC  Connectors=on both sides  ID=834  Vbase=Vnom  Vref=[1.0309 1.0295 1.0313]  Vangle=[-3.24 -124.39 116.09]  VLF=1  VLFb=1  VLFc=1  angleLF=0  angleLFb=0  angleLFc=0
      settings: AttributesFormatString=%<ID>
  Load Flow Bus25 : powerlib/Measurements/Load Flow Bus  LConnTagsString=a|b|c  RConnTagsString=a|b|c  Phases=ABC  Connectors=on both sides  ID=860  Vbase=Vnom  Vref=[1.0305 1.0291 1.031]  Vangle=[-3.24 -124.39 116.09]  VLF=1  VLFb=1  VLFc=1  angleLF=0  angleLFb=0  angleLFc=0
      settings: AttributesFormatString=%<ID>
  Load Flow Bus26 : powerlib/Measurements/Load Flow Bus  LConnTagsString=a|b|c  RConnTagsString=a|b|c  Phases=ABC  Connectors=on both sides  ID=836  Vbase=Vnom  Vref=[1.0303 1.0287 1.0308]  Vangle=[-3.23 -124.39 116.09]  VLF=1  VLFb=1  VLFc=1  angleLF=0  angleLFb=0  angleLFc=0
      settings: AttributesFormatString=%<ID>
  Load Flow Bus27 : powerlib/Measurements/Load Flow Bus  LConnTagsString=a|b|c  RConnTagsString=a|b|c  Phases=ABC  Connectors=on both sides  ID=840  Vbase=Vnom  Vref=[1.0303 1.0287 1.0308]  Vangle=[-3.23 -124.39 116.09]  VLF=1  VLFb=1  VLFc=1  angleLF=0  angleLFb=0  angleLFc=0
      settings: AttributesFormatString=%<ID>
  Load Flow Bus29 : powerlib/Measurements/Load Flow Bus  LConnTagsString=a  Phases=B  Connectors=on one side  ID=838  Vbase=Vnom  Vref=1.0285  Vangle=-124.39  VLF=1  VLFb=1  VLFc=1  angleLF=0  angleLFb=0  angleLFc=0
      settings: AttributesFormatString=%<ID>
  Load Flow Bus3 : powerlib/Measurements/Load Flow Bus  LConnTagsString=a|b|c  RConnTagsString=a|b|c  Phases=ABC  Connectors=on both sides  ID=808  Vbase=Vnom  Vref=[1.0136 1.0296 1.0289]  Vangle=[-0.75 -120.95 119.3]  VLF=1  VLFb=1  VLFc=1  angleLF=0  angleLFb=0  angleLFc=0
      settings: AttributesFormatString=%<ID>
  Load Flow Bus30 : powerlib/Measurements/Load Flow Bus  LConnTagsString=a|b|c  RConnTagsString=a|b|c  Phases=ABC  Connectors=on both sides  ID=842  Vbase=Vnom  Vref=[1.0309 1.0294 1.0313]  Vangle=[-3.25 -124.39 116.09]  VLF=1  VLFb=1  VLFc=1  angleLF=0  angleLFb=0  angleLFc=0
      settings: AttributesFormatString=%<ID>
  Load Flow Bus31 : powerlib/Measurements/Load Flow Bus  LConnTagsString=a|b|c  RConnTagsString=a|b|c  Phases=ABC  Connectors=on both sides  ID=844  Vbase=Vnom  Vref=[1.0307 1.0291 1.0311]  Vangle=[-3.27 -124.42 116.06]  VLF=1  VLFb=1  VLFc=1  angleLF=0  angleLFb=0  angleLFc=0
      settings: AttributesFormatString=%<ID>
  Load Flow Bus32 : powerlib/Measurements/Load Flow Bus  LConnTagsString=a|b|c  RConnTagsString=a|b|c  Phases=ABC  Connectors=on both sides  ID=846  Vbase=Vnom  Vref=[1.0309 1.0291 1.0313]  Vangle=[-3.32 -124.46 116.01]  VLF=1  VLFb=1  VLFc=1  angleLF=0  angleLFb=0  angleLFc=0
      settings: AttributesFormatString=%<ID>
  Load Flow Bus33 : powerlib/Measurements/Load Flow Bus  LConnTagsString=a|b|c  RConnTagsString=a|b|c  Phases=ABC  Connectors=on both sides  ID=848  Vbase=Vnom  Vref=[1.031 1.0291 1.0314]  Vangle=[-3.32 -124.47 116]  VLF=1  VLFb=1  VLFc=1  angleLF=0  angleLFb=0  angleLFc=0
      settings: AttributesFormatString=%<ID>
  Load Flow Bus34 : powerlib/Measurements/Load Flow Bus  LConnTagsString=a  Phases=A  Connectors=on one side  ID=open862  Vbase=Vnom  Vref=1.0303  Vangle=-3.23  VLF=1  VLFb=1  VLFc=1  angleLF=0  angleLFb=0  angleLFc=0
      settings: AttributesFormatString=%<ID>
  Load Flow Bus35 : powerlib/Measurements/Load Flow Bus  LConnTagsString=a  Phases=C  Connectors=on one side  ID=open862  Vbase=Vnom  Vref=1.0308  Vangle=116.09  VLF=1  VLFb=1  VLFc=1  angleLF=0  angleLFb=0  angleLFc=0
      settings: AttributesFormatString=%<ID>
  Load Flow Bus36 : powerlib/Measurements/Load Flow Bus  LConnTagsString=a  RConnTagsString=a  Phases=B  Connectors=on both sides  ID=862  Vbase=Vnom  Vref=1.0287  Vangle=-124.39  VLF=1  VLFb=1  VLFc=1  angleLF=0  angleLFb=0  angleLFc=0
      settings: AttributesFormatString=%<ID>
  Load Flow Bus4 : powerlib/Measurements/Load Flow Bus  LConnTagsString=a|b|c  RConnTagsString=a|b|c  Phases=ABC  Connectors=on both sides  ID=812  Vbase=Vnom  Vref=[0.9763 1.01 1.0069]  Vangle=[-1.57 -121.92 118.59]  VLF=1  VLFb=1  VLFc=1  angleLF=0  angleLFb=0  angleLFc=0
      settings: AttributesFormatString=%<ID>
  Load Flow Bus5 : powerlib/Measurements/Load Flow Bus  LConnTagsString=a|b|c  RConnTagsString=a|b|c  Phases=ABC  Connectors=on both sides  ID=814  Vbase=Vnom  Vref=[0.9467 0.9945 0.9893]  Vangle=[-2.26 -122.7 118.01]  VLF=1  VLFb=1  VLFc=1  angleLF=0  angleLFb=0  angleLFc=0
      settings: AttributesFormatString=%<ID>
  Load Flow Bus6 : powerlib/Measurements/Load Flow Bus  LConnTagsString=a  Phases=B  Connectors=on one side  ID=810  Vbase=Vnom  Vref=1.0294  Vangle=-120.95  VLF=1  VLFb=1  VLFc=1  angleLF=0  angleLFb=0  angleLFc=0
      settings: AttributesFormatString=%<ID>
  Load Flow Bus7 : powerlib/Measurements/Load Flow Bus  LConnTagsString=a|b|c  RConnTagsString=a|b|c  Phases=ABC  Connectors=on both sides  ID=850  Vbase=Vnom  Vref=[1.0176 1.0255 1.0203]  Vangle=[-2.26 -122.7 118.01]  VLF=1  VLFb=1  VLFc=1  angleLF=0  angleLFb=0  angleLFc=0
      settings: AttributesFormatString=%<ID>
  Load Flow Bus8 : powerlib/Measurements/Load Flow Bus  LConnTagsString=a|b|c  RConnTagsString=a|b|c  Phases=ABC  Connectors=on both sides  ID=816  Vbase=Vnom  Vref=[1.0172 1.0253 1.02]  Vangle=[-2.26 -122.71 1.02]  VLF=1  VLFb=1  VLFc=1  angleLF=0  angleLFb=0  angleLFc=0
      settings: AttributesFormatString=%<ID>
  Load Flow Bus9 : powerlib/Measurements/Load Flow Bus  LConnTagsString=a|b|c  RConnTagsString=a|b|c  Phases=ABC  Connectors=on both sides  ID=824  Vbase=Vnom  Vref=[1.0082 1.0158 1.0116]  Vangle=[-2.37 -122.94 117.76]  VLF=1  VLFb=1  VLFc=1  angleLF=0  angleLFb=0  angleLFc=0
      settings: AttributesFormatString=%<ID>
  MultiStateImage : MultiStateImageBlock  ScaleMode=Fill
  Power-Flow : Subsystem
      mask Display: disp('Power-Flow\nResults')
  XF-10 24.9kV / 4.16kV : powerlib/Elements/Three-Phase Transformer (Two Windings)  Winding1Connection=Yg  Winding2Connection=Yg  CoreType=Three single-phase transformers  SetSaturation=off  Hysteresis=off  DataFile='hysteresis'  SetInitialFlux=off  Measurements=None  UNITS=pu  NominalPower=[ 500e3 , 60 ]  Winding1=[ 24.9e3 , 0.019 , 0.0408 ]  Winding2=[ 4.16e3 , 0 , 0 ]  Rm=500  Lm=500  L0=0.5  Saturation=[ 0,0 ; 0.0024,1.2 ; 1.0,1.52 ]  InitialFluxes=[ 0.8 , -0.8 , 0.7 ]  BreakLoop=off  DiscreteSolver=Trapezoidal iterative  DataType=off  TransfoNumber=1
  powergui : powerlib/powergui  Priority=1  SimulationMode=Phasor  SampleTime=50e-6  frequency=60  Iterations=50  frequencyindice=60  Pbase=100e3  ErrMax=0.0001  UnitsV=kV  UnitsW=kW  buscounter=0  FunctionMessages=off  echomessages=off  EnableUseOfTLC=off  CurrentSourceSwitches=off  DisableSnubberDevices=off  DisableRonSwitches=off  DisableVfSwitches=off  DisplayEquations=off  AutomaticDiscreteSolvers=off  SolverType=Tustin/Backward Euler (TBE)  Interpol=off  ExternalGateDelay=off  methode=off  Ts=100  x0status=blocks  SPID=off  SwTol=0  HookPort=off  NonlinearTolerance=1e-4  nMaxIteration=100  ContinueOnMaxIteration=off  RestoreLinks=warning  ResistiveCurrentMeasurement=off  Frange=[0:2:500]  Ylog=off  Xlog=on  ShowGrid=off  save=off  variable=ZData  structure=0  ZoomFFT=on  StartTime=0.0  cycles=1  DisplayStyle=1  fundamental=60  FreqAxis=off  MaxFrequency=1000  frequencyindicesteady=1  RmsSteady=1  display=off
  wires:
  Constant3/1 -> Breaker832-858/1
  Constant5/1 -> Breaker836-862/1
  Constant4/1 -> Breaker834-842/1
  Constant1/1 -> Breaker850-816/1
  Constant2/1 -> Breaker818-820/1
  connections:
  800-802/RConn1 -- Load Flow Bus1/LConn1
  800-802/RConn2 -- Load Flow Bus1/LConn2
  800-802/RConn3 -- Load Flow Bus1/LConn3
  802/LConn1 -- Load Flow Bus1/RConn1
  802/LConn2 -- Load Flow Bus1/RConn2
  802/LConn3 -- Load Flow Bus1/RConn3
  802-806/LConn1 -- 802/RConn1 -- 802 Yg PQ/LConn1
  802-806/LConn2 -- 802/RConn2 -- 802 Yg PQ/LConn2
  802-806/LConn3 -- 802/RConn3 -- 802 Yg PQ/LConn3
  Load Flow Bus2/LConn1 -- 802-806/RConn1 -- 806 Yg PQ/LConn1
  Load Flow Bus2/LConn2 -- 802-806/RConn2 -- 806 Yg PQ/LConn2
  Load Flow Bus2/LConn3 -- 806 Yg PQ/LConn3 -- 802-806/RConn3
  808/LConn2 -- Load Flow Bus3/RConn2
  808/LConn3 -- Load Flow Bus3/RConn3
  Load Flow Bus3/LConn3 -- 806-808/RConn3
  Load Flow Bus3/LConn1 -- 806-808/RConn1
  Load Flow Bus3/LConn2 -- 806-808/RConn2
  808/LConn1 -- Load Flow Bus3/RConn1
  Load Flow Bus4/LConn3 -- 808-812/RConn3
  Load Flow Bus4/LConn1 -- 808-812/RConn1
  Load Flow Bus4/LConn2 -- 808-812/RConn2
  808-812/LConn1 -- 808/RConn1
  808-812/LConn2 -- 808 Y-I/LConn1 -- 808-810/LConn1 -- 808/RConn2
  808-812/LConn3 -- 808/RConn3
  Load Flow Bus5/LConn3 -- 812-814/RConn3
  Load Flow Bus5/LConn1 -- 812-814/RConn1
  Load Flow Bus5/LConn2 -- 812-814/RConn2
  Load Flow Bus7/LConn1 -- 814-850/RConn1
  Load Flow Bus7/LConn2 -- 814-850/RConn2
  Load Flow Bus7/LConn3 -- 814-850/RConn3
  816/LConn3 -- Load Flow Bus8/RConn3
  816/LConn1 -- Load Flow Bus8/RConn1
  816/LConn2 -- Load Flow Bus8/RConn2
  Load Flow Bus8/LConn2 -- 850-816/RConn2
  Load Flow Bus8/LConn3 -- 850-816/RConn3
  Load Flow Bus8/LConn1 -- 850-816/RConn1
  Load Flow Bus9/LConn2 -- 824 D-I/LConn2 -- 816-824/RConn2
  824/LConn1 -- Load Flow Bus9/RConn1
  Load Flow Bus9/LConn1 -- 824 D-I/LConn1 -- 816-824/RConn1
  824/LConn2 -- Load Flow Bus9/RConn2
  824/LConn3 -- Load Flow Bus9/RConn3
  Load Flow Bus9/LConn3 -- 824 D-I/LConn3 -- 816-824/RConn3
  816-824/LConn1 -- 816-818/LConn1 -- 816 D-I/LConn1 -- 816/RConn1
  816-824/LConn2 -- 816 D-I/LConn2 -- 816/RConn2
  816-824/LConn3 -- 816 D-I/LConn3 -- 816/RConn3
  824-828/LConn1 -- 824 Y-PQ/LConn1 -- 824/RConn1
  824-828/LConn2 -- 824 Y-PQ/LConn2 -- 824-826/LConn1 -- 824 Y-I/LConn1 -- 824/RConn2
  824-828/LConn3 -- 824 Y-PQ/LConn3 -- 824/RConn3
  818-820/LConn1 -- Breaker818-820/RConn1 -- 818 Y-Z/LConn1
  820-822/LConn1 -- 820/RConn1 -- 820 Y-PQ/LConn1
  820 Y-Z/LConn1 -- 818-820/RConn1 -- Load Flow Bus12/LConn1
  822 Y-PQ/LConn1 -- 822/RConn1 -- Load Flow Bus13/LConn1
  828/LConn2 -- Load Flow Bus14/RConn2
  Load Flow Bus14/LConn3 -- 824-828/RConn3 -- 828 Y-PQ/LConn3
  828/LConn1 -- Load Flow Bus14/RConn1
  Load Flow Bus14/LConn1 -- 828 Y-PQ/LConn1 -- 824-828/RConn1
  828/LConn3 -- Load Flow Bus14/RConn3
  Load Flow Bus14/LConn2 -- 824-828/RConn2 -- 828 Y-PQ/LConn2
  830 Y-PQ/LConn1 -- Load Flow Bus15/LConn1 -- 828-830/RConn1
  830 Y-PQ/LConn2 -- Load Flow Bus15/LConn2 -- 828-830/RConn2
  830 Y-PQ/LConn3 -- Load Flow Bus15/LConn3 -- 828-830/RConn3
  828-830/LConn1 -- 828 Y-PQ1/LConn1 -- 828/RConn1
  828-830/LConn2 -- 828 Y-PQ1/LConn2 -- 828/RConn2
  828-830/LConn3 -- 828 Y-PQ1/LConn3 -- 828/RConn3
  Load Flow Bus16/LConn1 -- 830-854/RConn1
  Load Flow Bus16/LConn2 -- 830-854/RConn2
  Load Flow Bus16/LConn3 -- 830-854/RConn3
  Load Flow Bus19/LConn3 -- 852-832/RConn3
  Load Flow Bus19/LConn2 -- 852-832/RConn2
  832/LConn1 -- Load Flow Bus19/RConn1
  Load Flow Bus19/LConn1 -- 852-832/RConn1
  832/LConn2 -- Load Flow Bus19/RConn2
  832/LConn3 -- Load Flow Bus19/RConn3
  854 Y-PQ/LConn1 -- 854-852/LConn2 -- 854/RConn2 -- 854-856/LConn1
  890/LConn1 -- Load Flow Bus21/RConn1
  890/LConn2 -- Load Flow Bus21/RConn2
  Load Flow Bus21/LConn1 -- 888-890/RConn1
  Load Flow Bus21/LConn2 -- 888-890/RConn2
  890/LConn3 -- Load Flow Bus21/RConn3
  Load Flow Bus21/LConn3 -- 888-890/RConn3
  890 D-I/LConn1 -- 890/RConn1
  890 D-I/LConn2 -- 890/RConn2
  890 D-I/LConn3 -- 890/RConn3
  858-834/LConn2 -- 858 D-PQ/LConn2 -- 858/RConn2
  Load Flow Bus22/LConn3 -- 858 D-Z/LConn3 -- 832-858/RConn3
  Load Flow Bus22/LConn1 -- 858 D-Z/LConn1 -- 832-858/RConn1
  858/LConn3 -- Load Flow Bus22/RConn3
  Load Flow Bus22/LConn2 -- 858 D-Z/LConn2 -- 832-858/RConn2
  858/LConn1 -- Load Flow Bus22/RConn1
  858-834/LConn1 -- 858 D-PQ/LConn1 -- 858-864/LConn1 -- 858 Y-PQ/LConn1 -- 858/RConn1
  858/LConn2 -- Load Flow Bus22/RConn2
  858-834/LConn3 -- 858 D-PQ/LConn3 -- 858/RConn3
  Load Flow Bus25/LConn3 -- 860 D-Z/LConn3 -- 834-860/RConn3
  834-860/LConn1 -- 834 D-Z/LConn1 -- Breaker834-842/RConn1 -- 834/RConn1
  834/LConn2 -- Load Flow Bus24/RConn2
  860/LConn3 -- Load Flow Bus25/RConn3
  834/LConn3 -- Load Flow Bus24/RConn3
  860/LConn1 -- Load Flow Bus25/RConn1
  Load Flow Bus24/LConn2 -- 834 D-PQ/LConn2 -- 858-834/RConn2
  Load Flow Bus24/LConn1 -- 834 D-PQ/LConn1 -- 858-834/RConn1
  Load Flow Bus24/LConn3 -- 834 D-PQ/LConn3 -- 858-834/RConn3
  834/LConn1 -- Load Flow Bus24/RConn1
  Load Flow Bus25/LConn2 -- 860 D-Z/LConn2 -- 834-860/RConn2
  860/LConn2 -- Load Flow Bus25/RConn2
  834-860/LConn3 -- 834 D-Z/LConn3 -- Breaker834-842/RConn3 -- 834/RConn3
  834-860/LConn2 -- 834 D-Z/LConn2 -- Breaker834-842/RConn2 -- 834/RConn2
  Load Flow Bus25/LConn1 -- 860 D-Z/LConn1 -- 834-860/RConn1
  XF-10 24.9kV / 4.16kV/LConn1 -- 832/RConn1 -- Breaker832-858/RConn1
  XF-10 24.9kV / 4.16kV/LConn2 -- 832/RConn2 -- Breaker832-858/RConn2
  832 D-Z/LConn3 -- 832-858/LConn3 -- Breaker832-858/LConn3
  Load Flow Bus26/LConn1 -- 836 D-PQ/LConn1 -- 860-836/RConn1
  Load Flow Bus26/LConn2 -- 836 D-PQ/LConn2 -- 860-836/RConn2
  836/LConn3 -- Load Flow Bus26/RConn3
  836/LConn1 -- Load Flow Bus26/RConn1
  Load Flow Bus26/LConn3 -- 836 D-PQ/LConn3 -- 860-836/RConn3
  836/LConn2 -- Load Flow Bus26/RConn2
  860-836/LConn1 -- 860 D-PQ/LConn1 -- 860 Y-PQ/LConn1 -- 860/RConn1
  860-836/LConn2 -- 860 D-PQ/LConn2 -- 860 Y-PQ/LConn2 -- 860/RConn2
  860-836/LConn3 -- 860 D-PQ/LConn3 -- 860 Y-PQ/LConn3 -- 860/RConn3
  Load Flow Bus27/LConn1 -- 836-840/RConn1 -- 840 D-I/LConn1
  Load Flow Bus27/LConn2 -- 836-840/RConn2 -- 840 D-I/LConn2
  840/LConn1 -- Load Flow Bus27/RConn1
  840/LConn2 -- Load Flow Bus27/RConn2
  Load Flow Bus27/LConn3 -- 836-840/RConn3 -- 840 D-I/LConn3
  840/LConn3 -- Load Flow Bus27/RConn3
  836-840/LConn1 -- Breaker836-862/LConn1 -- 836/RConn1 -- 836 D-I/LConn1
  836-840/LConn2 -- Breaker836-862/LConn2 -- 836/RConn2 -- 836 D-I/LConn2
  836-840/LConn3 -- Breaker836-862/LConn3 -- 836/RConn3 -- 836 D-I/LConn3
  840 Y-I/LConn1 -- 840/RConn1
  840 Y-I/LConn2 -- 840/RConn2
  840 Y-I/LConn3 -- 840/RConn3
  Load Flow Bus30/LConn1 -- 834-842/RConn1
  842/LConn2 -- Load Flow Bus30/RConn2
  842/LConn3 -- Load Flow Bus30/RConn3
  Load Flow Bus30/LConn2 -- 834-842/RConn2
  Load Flow Bus30/LConn3 -- 834-842/RConn3
  842/LConn1 -- Load Flow Bus30/RConn1
  Load Flow Bus31/LConn2 -- 844 Y-PQ/LConn2 -- 842-844/RConn2
  844/LConn2 -- Load Flow Bus31/RConn2
  Load Flow Bus31/LConn1 -- 844 Y-PQ/LConn1 -- 842-844/RConn1
  844/LConn1 -- Load Flow Bus31/RConn1
  842-844/LConn1 -- 842 Y-PQ/LConn1 -- 842/RConn1
  842-844/LConn2 -- 842 Y-PQ/LConn2 -- 842/RConn2
  842-844/LConn3 -- 842 Y-PQ/LConn3 -- 842/RConn3
  Load Flow Bus32/LConn2 -- 844-846/RConn2 -- 846 Y-PQ/LConn2
  846/LConn2 -- Load Flow Bus32/RConn2
  Load Flow Bus32/LConn1 -- 844-846/RConn1 -- 846 Y-PQ/LConn1
  846/LConn1 -- Load Flow Bus32/RConn1
  844-846/LConn1 -- 844 Y-PQ1/LConn1 -- 844 Y-Z1/LConn1 -- 844 Y-Z/LConn1 -- 844/RConn1
  844-846/LConn2 -- 844 Y-PQ1/LConn2 -- 844 Y-Z1/LConn2 -- 844 Y-Z/LConn2 -- 844/RConn2
  844-846/LConn3 -- 844 Y-PQ1/LConn3 -- 844 Y-Z1/LConn3 -- 844 Y-Z/LConn3 -- 844/RConn3
  Load Flow Bus33/LConn2 -- 848 Y-PQ/LConn2 -- 846-848/RConn2
  848/LConn2 -- Load Flow Bus33/RConn2
  Load Flow Bus33/LConn1 -- 848 Y-PQ/LConn1 -- 846-848/RConn1
  848/LConn1 -- Load Flow Bus33/RConn1
  846-848/LConn1 -- 846 Y-PQ1/LConn1 -- 846/RConn1
  846-848/LConn2 -- 846 Y-PQ1/LConn2 -- 846/RConn2
  846-848/LConn3 -- 846 Y-PQ1/LConn3 -- 846/RConn3
  848 D-PQ/LConn1 -- 848 D-Z/LConn1 -- 848/RConn1
  848 D-PQ/LConn2 -- 848 D-Z/LConn2 -- 848/RConn2
  848 D-PQ/LConn3 -- 848 D-Z/LConn3 -- 848/RConn3
  Load Flow Bus20/LConn1 -- XF-10 24.9kV / 4.16kV/RConn1
  Load Flow Bus20/LConn2 -- XF-10 24.9kV / 4.16kV/RConn2
  Load Flow Bus20/LConn3 -- XF-10 24.9kV / 4.16kV/RConn3
  826 Y-I/LConn1 -- 826/RConn2 -- Load Flow Bus10/LConn1
  838 Y-PQ/LConn1 -- 838/RConn2 -- Load Flow Bus29/LConn1
  Ground1/LConn1 -- 810 Y-I/RConn1
  Ground2/LConn1 -- 818 Y-Z/RConn1
  Ground3/LConn1 -- 820 Y-Z/RConn1
  Ground4/LConn1 -- 820 Y-PQ/RConn1
  Ground5/LConn1 -- 822 Y-PQ/RConn1
  862-838/LConn1 -- 862 Y-PQ/LConn1 -- Load Flow Bus36/RConn1
  Ground8/LConn1 -- 824 Y-I/RConn1
  Ground9/LConn1 -- 826 Y-I/RConn1
  842-844/RConn3 -- 844 Y-PQ/LConn3 -- Load Flow Bus31/LConn3
  Load Flow Bus31/RConn3 -- 844/LConn3
  844-846/RConn3 -- 846 Y-PQ/LConn3 -- Load Flow Bus32/LConn3
  Load Flow Bus32/RConn3 -- 846/LConn3
  846-848/RConn3 -- 848 Y-PQ/LConn3 -- Load Flow Bus33/LConn3
  Load Flow Bus33/RConn3 -- 848/LConn3
  Ground10/LConn1 -- 854 Y-PQ/RConn1
  Ground11/LConn1 -- 856 Y-PQ/RConn1
  Ground12/LConn1 -- 858 Y-PQ/RConn1
  Ground13/LConn1 -- 864 Y-PQ/RConn1
  864 Y-PQ/LConn1 -- 864/RConn1 -- Load Flow Bus23/LConn1
  Ground14/LConn1 -- 862 Y-PQ/RConn1
  Ground15/LConn1 -- 838 Y-PQ/RConn1
  Load Flow Bus/RConn1 -- 800-802/LConn1
  Load Flow Bus/RConn2 -- 800-802/LConn2
  Load Flow Bus/RConn3 -- 800-802/LConn3
  830/LConn1 -- Load Flow Bus15/RConn1
  830/LConn2 -- Load Flow Bus15/RConn2
  830/LConn3 -- Load Flow Bus15/RConn3
  830-854/LConn1 -- 830 D-Z/LConn1 -- 830/RConn1
  830-854/LConn2 -- 830 D-Z/LConn2 -- 830/RConn2
  830-854/LConn3 -- 830 D-Z/LConn3 -- 830/RConn3
  810/LConn2 -- 808-810/RConn1
  816-818/RConn1 -- Load Flow Bus11/LConn1
  832 D-Z/LConn1 -- 832-858/LConn1 -- Breaker832-858/LConn1
  XF-10 24.9kV / 4.16kV/LConn3 -- Breaker832-858/RConn3 -- 832/RConn3
  832 D-Z/LConn2 -- 832-858/LConn2 -- Breaker832-858/LConn2
  Ground/LConn1 -- 808 Y-I/RConn1
  Breaker836-862/RConn1 -- 836-862/LConn1
  Breaker836-862/RConn2 -- 836-862/LConn2
  Breaker836-862/RConn3 -- 836-862/LConn3
  834-842/LConn1 -- Breaker834-842/LConn1
  834-842/LConn2 -- Breaker834-842/LConn2
  834-842/LConn3 -- Breaker834-842/LConn3
  Breaker850-816/LConn3 -- 850-816/LConn1
  Breaker850-816/LConn2 -- 850-816/LConn2
  Breaker850-816/LConn1 -- 850-816/LConn3
  818/LConn1 -- Load Flow Bus11/RConn1
  818/RConn1 -- Breaker818-820/LConn1
  818/RConn2 -- 818/RConn3 -- 818/LConn3 -- 818/LConn2 -- Ground6/LConn1
  806/RConn1 -- 806-808/LConn1
  806/LConn1 -- Load Flow Bus2/RConn1
  806/LConn2 -- Load Flow Bus2/RConn2
  806/RConn2 -- 806-808/LConn2
  806/RConn3 -- 806-808/LConn3
  806/LConn3 -- Load Flow Bus2/RConn3
  812/RConn1 -- 812-814/LConn1
  812/LConn1 -- Load Flow Bus4/RConn1
  812/LConn2 -- Load Flow Bus4/RConn2
  812/RConn2 -- 812-814/LConn2
  812/LConn3 -- Load Flow Bus4/RConn3
  812/RConn3 -- 812-814/LConn3
  814/RConn1 -- 814-850/LConn1
  814/LConn1 -- Load Flow Bus5/RConn1
  Load Flow Bus5/RConn2 -- 814/LConn2
  Load Flow Bus5/RConn3 -- 814/LConn3
  814/RConn2 -- 814-850/LConn2
  814-850/LConn3 -- 814/RConn3
  810/RConn3 -- 810/LConn1 -- 810/LConn3 -- Ground7/LConn1 -- 810/RConn1
  810/RConn2 -- 810 Y-I/LConn1 -- Load Flow Bus6/LConn1
  850/RConn1 -- Breaker850-816/RConn3
  850/RConn2 -- Breaker850-816/RConn2
  850/RConn3 -- Breaker850-816/RConn1
  850/LConn1 -- Load Flow Bus7/RConn1
  850/LConn2 -- Load Flow Bus7/RConn2
  850/LConn3 -- Load Flow Bus7/RConn3
  820/RConn2 -- 820/LConn3 -- 820/LConn2 -- Ground16/LConn1 -- 820/RConn3
  Load Flow Bus12/RConn1 -- 820/LConn1
  822/RConn2 -- 822/LConn3 -- 822/LConn2 -- Ground17/LConn1 -- 822/RConn3
  822/LConn1 -- 820-822/RConn1
  826/RConn3 -- 826/LConn1 -- 826/LConn3 -- Ground18/LConn1 -- 826/RConn1
  826/LConn2 -- 824-826/RConn1
  854/LConn1 -- Load Flow Bus16/RConn1
  854/LConn2 -- Load Flow Bus16/RConn2
  854/LConn3 -- Load Flow Bus16/RConn3
  856/LConn2 -- 854-856/RConn1
  852/RConn1 -- 852-832/LConn1
  852/RConn2 -- 852-832/LConn2
  852/RConn3 -- 852-832/LConn3
  888/LConn1 -- Load Flow Bus20/RConn1
  888/LConn2 -- Load Flow Bus20/RConn2
  888/LConn3 -- Load Flow Bus20/RConn3
  888/RConn1 -- 888-890/LConn1
  888/RConn2 -- 888-890/LConn2
  888/RConn3 -- 888-890/LConn3
  864/RConn3 -- 864/LConn2 -- 864/LConn3 -- Ground20/LConn1 -- 864/RConn2
  864/LConn1 -- 858-864/RConn1
  836-862/RConn1 -- 862/LConn1
  836-862/RConn2 -- 862/LConn2
  836-862/RConn3 -- 862/LConn3
  Load Flow Bus34/LConn1 -- 862/RConn1
  Load Flow Bus36/LConn1 -- 862/RConn2
  Load Flow Bus35/LConn1 -- 862/RConn3
  838/LConn3 -- 838/LConn1 -- 838/RConn1 -- 838/RConn3 -- Ground21/LConn1
  838/LConn2 -- 862-838/RConn1
  800 gen/RConn1 -- Load Flow Bus/LConn1
  800 gen/RConn2 -- Load Flow Bus/LConn2
  800 gen/RConn3 -- Load Flow Bus/LConn3
  856/LConn3 -- Ground19/LConn1 -- 856/RConn3 -- 856/RConn1 -- 856/LConn1
  856/RConn2 -- Load Flow Bus17/LConn1 -- 856 Y-PQ/LConn1
  Load Flow Bus18/RConn2 -- 852/LConn2
  Load Flow Bus18/RConn3 -- 852/LConn3
  Load Flow Bus18/RConn1 -- 852/LConn1
  854-852/RConn1 -- Load Flow Bus18/LConn1
  854-852/RConn2 -- Load Flow Bus18/LConn2
  854-852/RConn3 -- Load Flow Bus18/LConn3
  854/RConn1 -- 854-852/LConn1
  854/RConn3 -- 854-852/LConn3
